simulink model "full_simulation_split_hil_new_connection"  (Simulink 7.9)
settings: Solver=ode1  StartTime=0  StopTime=10  FixedStep=Ts  RelTol=1e-8
values from neighbouring files (symbols this model uses):
  A_fx = 2e-2 * 0.4    (= 0.008)    [QR_DI_Init.m]    (also in quadro_cascade_disturbance_wo_wind.m)
  A_fy = A_fx    (= 0.008)    [QR_DI_Init.m]    (also in quadro_cascade_disturbance_wo_wind.m)
  A_fz = 2 * A_fx    (= 0.016)    [QR_DI_Init.m]    (also in quadro_cascade_disturbance_wo_wind.m)
  Bias_Phi = -0.0088    [QR_DI_Init.m]    (also in Reference_Calibration.m = mean(Phi))
  Bias_Theta = 0.022    [QR_DI_Init.m]    (also in Reference_Calibration.m = mean(Theta))
  command_on = 1    [QR_DI_Init.m]    (also in quadro_cascade_disturbance_wo_wind.m)
  cw_x = 1.05    [QR_DI_Init.m]    (also in quadro_cascade_disturbance_wo_wind.m)
  cw_y = cw_x    (= 1.05)    [QR_DI_Init.m]    (also in quadro_cascade_disturbance_wo_wind.m)
  cw_z = 1.05    [QR_DI_Init.m]    (also in quadro_cascade_disturbance_wo_wind.m)
  deltaTm = 0.2    [QR_DI_Init.m]    (also in quadro_cascade_disturbance_wo_wind.m)
  den_psi_ref = poly( ones(1,2) * -1 * T_psi_ref)    [QR_DI_Init.m]    (also in quadro_cascade_disturbance_wo_wind.m)
  den_x_ref = poly( ones(1,4) * -1 * T_x_ref)    [QR_DI_Init.m]    (also in quadro_cascade_disturbance_wo_wind.m)
  den_y_ref = poly( ones(1,4) * -1 * T_y_ref)    [QR_DI_Init.m]    (also in quadro_cascade_disturbance_wo_wind.m)
  den_z_ref = poly( ones(1,4) * -1 * T_z_ref)    [QR_DI_Init.m]    (also in quadro_cascade_disturbance_wo_wind.m)
  drot = 0.0117    [QR_DI_Init.m]    (also in quadro_cascade_disturbance_wo_wind.m = 0.2)
  dtran = 0.01    [QR_DI_Init.m]    (also in quadro_cascade_disturbance_wo_wind.m = 0.003)
  Fz_gain = 1 + 0.05*rand(1)    [QR_DI_Init.m]    (also in quadro_cascade_disturbance_wo_wind.m)
  Fz_lo = - 1.2 * m * g    (= -3.5316)    [QR_DI_Init.m]    (also in quadro_cascade_disturbance_wo_wind.m = -4.1202)
  Fz_up = 0    [QR_DI_Init.m]    (also in quadro_cascade_disturbance_wo_wind.m)
  g = 9.81    [QR_DI_Init.m]    (also in quadro_cascade_disturbance_wo_wind.m)
  Iq = [I_xx 0 0 ; 0 I_yy 0 ; 0 0 I_zz ]    [QR_DI_Init.m]    (also in quadro_cascade_disturbance_wo_wind.m = [0.0605 0 0; 0 0.0605 0; 0 0 0.018])
  K_err = old(:,2:end)    [QR_DI_Init.m]    (also in quadro_cascade_disturbance_wo_wind.m)
  K_Mot_Force = 0.3512    [QR_DI_Init.m]    (also in quadro_cascade_disturbance_wo_wind.m)
  K_Mot_Torque = 0.013    [QR_DI_Init.m]    (also in quadro_cascade_disturbance_wo_wind.m = 0.0013)
  l = 0.25    [QR_DI_Init.m]    (also in quadro_cascade_disturbance_wo_wind.m = 0.2775)
  m = 0.30    (= 0.3)    [QR_DI_Init.m]    (also in quadro_cascade_disturbance_wo_wind.m)
  m_real = m * ( 1 + 0.05*rand(1))    [QR_DI_Init.m]    (also in quadro_cascade_disturbance_wo_wind.m)
  Mm = 0.0    (= 0)    [QR_DI_Init.m]    (also in quadro_cascade_disturbance_wo_wind.m = 0.5)
  Mx_lo = - Mx_up    (= -0.2)    [QR_DI_Init.m]    (also in quadro_cascade_disturbance_wo_wind.m)
  Mx_up = 0.20    (= 0.2)    [QR_DI_Init.m]    (also in quadro_cascade_disturbance_wo_wind.m)
  My_lo = - My_up    (= -0.2)    [QR_DI_Init.m]    (also in quadro_cascade_disturbance_wo_wind.m)
  My_up = 0.20    (= 0.2)    [QR_DI_Init.m]    (also in quadro_cascade_disturbance_wo_wind.m)
  Mz_lo = - Mz_up    (= -0.02)    [QR_DI_Init.m]    (also in quadro_cascade_disturbance_wo_wind.m = -0.002)
  Mz_up = 0.02    [QR_DI_Init.m]    (also in quadro_cascade_disturbance_wo_wind.m = 0.002)
  phase_wind_z = 0    [QR_DI_Init.m]    (also in quadro_cascade_disturbance_wo_wind.m)
  psi_p_lim = 10*pi/180    (= 0.174532925199)    [QR_DI_Init.m]    (also in quadro_cascade_disturbance_wo_wind.m = 5)
  PWM_MAX = 200    [QR_DI_Init.m]    (also in quadro_cascade_disturbance_wo_wind.m)
  rho_air = 1.2041    [QR_DI_Init.m]    (also in quadro_cascade_disturbance_wo_wind.m)
  sample_time_noise_psi = 0.1    [QR_DI_Init.m]
  sample_time_noise_x = 0.2    [QR_DI_Init.m]
  sample_time_noise_y = 0.2    [QR_DI_Init.m]
  sample_time_noise_z = 0.1    [QR_DI_Init.m]
  seed_psi = seedvector(7)    [QR_DI_Init.m]
  seed_x = seedvector(1)    [QR_DI_Init.m]    (also in quadro_cascade_disturbance_wo_wind.m)
  seed_xp = seedvector(4)    [QR_DI_Init.m]    (also in quadro_cascade_disturbance_wo_wind.m)
  seed_y = seedvector(2)    [QR_DI_Init.m]    (also in quadro_cascade_disturbance_wo_wind.m)
  seed_yp = seedvector(5)    [QR_DI_Init.m]    (also in quadro_cascade_disturbance_wo_wind.m)
  seed_z = seedvector(3)    [QR_DI_Init.m]    (also in quadro_cascade_disturbance_wo_wind.m)
  seed_zp = seedvector(6)    [QR_DI_Init.m]    (also in quadro_cascade_disturbance_wo_wind.m)
  std_dev_psi = 1 * pi/180 * Noise_on    (= 0)    [QR_DI_Init.m]
  std_dev_x = 1e-1 * Noise_on    (= 0)    [QR_DI_Init.m]
  std_dev_xp = 0.03 * Noise_on    (= 0)    [QR_DI_Init.m]
  std_dev_y = 1e-1 * Noise_on    (= 0)    [QR_DI_Init.m]
  std_dev_yp = 0.03 * Noise_on    (= 0)    [QR_DI_Init.m]
  std_dev_z = 0.03 * Noise_on    (= 0)    [QR_DI_Init.m]
  std_dev_zp = 0.03 * Noise_on    (= 0)    [QR_DI_Init.m]
  T_refalt = 0.01    [QR_DI_Init.m]    (also in quadro_cascade_disturbance_wo_wind.m)
  T_wind_z = 24    [QR_DI_Init.m]    (also in quadro_cascade_disturbance_wo_wind.m)
  Tm = 10    [QR_DI_Init.m]    (also in quadro_cascade_disturbance_wo_wind.m)
  Ts = 1e-2    (= 0.01)    [QR_DI_Init.m]    (also in quadro_cascade_disturbance_wo_wind.m)
  v_wind_max_z = 2    [QR_DI_Init.m]    (also in quadro_cascade_disturbance_wo_wind.m)
  wind_on = 0    [QR_DI_Init.m]    (also in quadro_cascade_disturbance_wo_wind.m)
  x_p_lim = 1.5    [QR_DI_Init.m]    (also in quadro_cascade_disturbance_wo_wind.m = 5)
  y_p_lim = 1.5    [QR_DI_Init.m]    (also in quadro_cascade_disturbance_wo_wind.m = 5)
  z_p_lim = 1    [QR_DI_Init.m]    (also in quadro_cascade_disturbance_wo_wind.m = 1.5)
undefined symbols (not defined in the file or in its folder): T_wind_fine, v_wind_x_fine, v_wind_y_fine
libraries: simulink x5, dspsigops x4, Ports x4, aerolibtransform2 x3, dspmtrx3 x1, aerolibutil x1
(part 4 of 6)

== matlab function Dynamic Inversion of the Extended System/bx1/Embedded MATLAB Function1 ==
  data: xwhole_ext input double size=[14 1]; bx output double size=[4 1]; m_in input double; I input double size=[3 3]; dtran input double; drot input double

% S.H. 26.03.2013
% correct bx

function bx = fcn(xwhole_ext, m_in, I, dtran, drot)
% This block supports the Embedded MATLAB subset.
% See the help menu for details. 
x = xwhole_ext(1);
y = xwhole_ext(2);
z = xwhole_ext(3);
dx = xwhole_ext(4);
dy = xwhole_ext(5);
dz = xwhole_ext(6);

phi = xwhole_ext(7);
theta = xwhole_ext(8);
psi = xwhole_ext(9);
p = xwhole_ext(10);
q = xwhole_ext(11);
r = xwhole_ext(12);


xi1 = xwhole_ext(13) +eps;
dxi1 = xwhole_ext(14) +eps;


%g = -9.81;
g = -9.81;   % S.H. 26.03.2013

m = m_in;

% FIXME: the bx is still the one without deviation components
Ixx = I(1,1);
Ixy = I(1,2);
Ixz = I(1,3);
Iyy = I(2,2);
Iyz = I(2,3);
Izz = I(3,3);

% S.H. 26.03.2013
bx =    [...
(p + r*cos(phi)*tan(theta) + q*sin(phi)*tan(theta))*((dxi1*(cos(phi)*sin(psi) - cos(psi)*sin(phi)*sin(theta)))/m - (xi1*(sin(phi)*sin(psi) + cos(phi)*cos(psi)*sin(theta))*(p + r*cos(phi)*tan(theta) + q*sin(phi)*tan(theta)))/m + (xi1*((r*cos(phi))/cos(theta) + (q*sin(phi))/cos(theta))*(cos(phi)*cos(psi) + sin(phi)*sin(psi)*sin(theta)))/m + (xi1*((q*cos(phi))/cos(theta) - (r*sin(phi))/cos(theta))*(cos(psi)*sin(phi) - cos(phi)*sin(psi)*sin(theta)))/m - (dtran*xi1*(cos(phi)*sin(psi) - cos(psi)*sin(phi)*sin(theta)))/m^2 + (xi1*(cos(phi)*sin(psi) - cos(psi)*sin(phi)*sin(theta))*(q*cos(phi)*tan(theta) - r*sin(phi)*tan(theta)))/m - (xi1*cos(phi)*cos(psi)*cos(theta)*(r*cos(phi) + q*sin(phi)))/m - (xi1*cos(psi)*cos(theta)*sin(phi)*(q*cos(phi) - r*sin(phi)))/m) - ((Ixx*p*r - Izz*p*r)/Iyy + (drot*q)/Iyy)*((xi1*sin(phi)*(cos(psi)*sin(phi) - cos(phi)*sin(psi)*sin(theta)))/(m*cos(theta)) + (xi1*cos(phi)^2*cos(psi)*cos(theta))/m + (xi1*sin(phi)*tan(theta)*(cos(phi)*sin(psi) - cos(psi)*sin(phi)*sin(theta)))/m) + ((Ixx*p*q - Iyy*p*q)/Izz - (drot*r)/Izz)*((xi1*cos(phi)*(cos(psi)*sin(phi) - cos(phi)*sin(psi)*sin(theta)))/(m*cos(theta)) + (xi1*cos(phi)*tan(theta)*(cos(phi)*sin(psi) - cos(psi)*sin(phi)*sin(theta)))/m - (xi1*cos(phi)*cos(psi)*cos(theta)*sin(phi))/m) - ((r*cos(phi))/cos(theta) + (q*sin(phi))/cos(theta))*((xi1*((r*cos(phi))/cos(theta) + (q*sin(phi))/cos(theta))*(sin(phi)*sin(psi) + cos(phi)*cos(psi)*sin(theta)))/m - (xi1*(cos(phi)*cos(psi) + sin(phi)*sin(psi)*sin(theta))*(p + r*cos(phi)*tan(theta) + q*sin(phi)*tan(theta)))/m - (dxi1*(cos(psi)*sin(phi) - cos(phi)*sin(psi)*sin(theta)))/m + (dtran*xi1*(cos(psi)*sin(phi) - cos(phi)*sin(psi)*sin(theta)))/m^2 + (xi1*cos(phi)*cos(theta)*sin(psi)*(q*cos(phi) - r*sin(phi)))/m) - (q*cos(phi) - r*sin(phi))*((xi1*cos(psi)*cos(theta)*sin(phi)*(p + r*cos(phi)*tan(theta) + q*sin(phi)*tan(theta)))/m - (xi1*(r*cos(phi)*(tan(theta)^2 + 1) + q*sin(phi)*(tan(theta)^2 + 1))*(cos(phi)*sin(psi) - cos(psi)*sin(phi)*sin(theta)))/m - (dxi1*cos(phi)*cos(psi)*cos(theta))/m - (xi1*(cos(psi)*sin(phi) - cos(phi)*sin(psi)*sin(theta))*((r*cos(phi)*sin(theta))/cos(theta)^2 + (q*sin(phi)*sin(theta))/cos(theta)^2))/m + (xi1*cos(phi)*cos(theta)*sin(psi)*((r*cos(phi))/cos(theta) + (q*sin(phi))/cos(theta)))/m + (dtran*xi1*cos(phi)*cos(psi)*cos(theta))/m^2 + (xi1*cos(phi)*cos(psi)*sin(theta)*(q*cos(phi) - r*sin(phi)))/m) + dxi1*(((cos(phi)*sin(psi) - cos(psi)*sin(phi)*sin(theta))*(p + r*cos(phi)*tan(theta) + q*sin(phi)*tan(theta)))/m - (dtran*(sin(phi)*sin(psi) + cos(phi)*cos(psi)*sin(theta)))/m^2 + (((r*cos(phi))/cos(theta) + (q*sin(phi))/cos(theta))*(cos(psi)*sin(phi) - cos(phi)*sin(psi)*sin(theta)))/m + (cos(phi)*cos(psi)*cos(theta)*(q*cos(phi) - r*sin(phi)))/m) + (dtran^2*((xi1*(sin(phi)*sin(psi) + cos(phi)*cos(psi)*sin(theta)))/m - (dtran*dx)/m))/m^2 + (xi1*(cos(phi)*sin(psi) - cos(psi)*sin(phi)*sin(theta))*((Iyy*q*r - Izz*q*r)/Ixx - (drot*p)/Ixx))/m;
        dxi1*((dtran*(cos(psi)*sin(phi) - cos(phi)*sin(psi)*sin(theta)))/m^2 - ((cos(phi)*cos(psi) + sin(phi)*sin(psi)*sin(theta))*(p + r*cos(phi)*tan(theta) + q*sin(phi)*tan(theta)))/m + (((r*cos(phi))/cos(theta) + (q*sin(phi))/cos(theta))*(sin(phi)*sin(psi) + cos(phi)*cos(psi)*sin(theta)))/m + (cos(phi)*cos(theta)*sin(psi)*(q*cos(phi) - r*sin(phi)))/m) - ((Ixx*p*r - Izz*p*r)/Iyy + (drot*q)/Iyy)*((xi1*sin(phi)*(sin(phi)*sin(psi) + cos(phi)*cos(psi)*sin(theta)))/(m*cos(theta)) + (xi1*cos(phi)^2*cos(theta)*sin(psi))/m - (xi1*sin(phi)*tan(theta)*(cos(phi)*cos(psi) + sin(phi)*sin(psi)*sin(theta)))/m) - (p + r*cos(phi)*tan(theta) + q*sin(phi)*tan(theta))*((dxi1*(cos(phi)*cos(psi) + sin(phi)*sin(psi)*sin(theta)))/m - (xi1*(cos(psi)*sin(phi) - cos(phi)*sin(psi)*sin(theta))*(p + r*cos(phi)*tan(theta) + q*sin(phi)*tan(theta)))/m - (xi1*((r*cos(phi))/cos(theta) + (q*sin(phi))/cos(theta))*(cos(phi)*sin(psi) - cos(psi)*sin(phi)*sin(theta)))/m - (xi1*((q*cos(phi))/cos(theta) - (r*sin(phi))/cos(theta))*(sin(phi)*sin(psi) + cos(phi)*cos(psi)*sin(theta)))/m - (dtran*xi1*(cos(phi)*cos(psi) + sin(phi)*sin(psi)*sin(theta)))/m^2 + (xi1*(cos(phi)*cos(psi) + sin(phi)*sin(psi)*sin(theta))*(q*cos(phi)*tan(theta) - r*sin(phi)*tan(theta)))/m + (xi1*cos(phi)*cos(theta)*sin(psi)*(r*cos(phi) + q*sin(phi)))/m + (xi1*cos(theta)*sin(phi)*sin(psi)*(q*cos(phi) - r*sin(phi)))/m) - ((Ixx*p*q - Iyy*p*q)/Izz - (drot*r)/Izz)*((xi1*cos(phi)*tan(theta)*(cos(phi)*cos(psi) + sin(phi)*sin(psi)*sin(theta)))/m - (xi1*cos(phi)*(sin(phi)*sin(psi) + cos(phi)*cos(psi)*sin(theta)))/(m*cos(theta)) + (xi1*cos(phi)*cos(theta)*sin(phi)*sin(psi))/m) + ((r*cos(phi))/cos(theta) + (q*sin(phi))/cos(theta))*((dxi1*(sin(phi)*sin(psi) + cos(phi)*cos(psi)*sin(theta)))/m + (xi1*(cos(phi)*sin(psi) - cos(psi)*sin(phi)*sin(theta))*(p + r*cos(phi)*tan(theta) + q*sin(phi)*tan(theta)))/m + (xi1*((r*cos(phi))/cos(theta) + (q*sin(phi))/cos(theta))*(cos(psi)*sin(phi) - cos(phi)*sin(psi)*sin(theta)))/m - (dtran*xi1*(sin(phi)*sin(psi) + cos(phi)*cos(psi)*sin(theta)))/m^2 + (xi1*cos(phi)*cos(psi)*cos(theta)*(q*cos(phi) - r*sin(phi)))/m) - (q*cos(phi) - r*sin(phi))*((xi1*(r*cos(phi)*(tan(theta)^2 + 1) + q*sin(phi)*(tan(theta)^2 + 1))*(cos(phi)*cos(psi) + sin(phi)*sin(psi)*sin(theta)))/m - (xi1*(sin(phi)*sin(psi) + cos(phi)*cos(psi)*sin(theta))*((r*cos(phi)*sin(theta))/cos(theta)^2 + (q*sin(phi)*sin(theta))/cos(theta)^2))/m - (dxi1*cos(phi)*cos(theta)*sin(psi))/m + (xi1*cos(theta)*sin(phi)*sin(psi)*(p + r*cos(phi)*tan(theta) + q*sin(phi)*tan(theta)))/m - (xi1*cos(phi)*cos(psi)*cos(theta)*((r*cos(phi))/cos(theta) + (q*sin(phi))/cos(theta)))/m + (dtran*xi1*cos(phi)*cos(theta)*sin(psi))/m^2 + (xi1*cos(phi)*sin(psi)*sin(theta)*(q*cos(phi) - r*sin(phi)))/m) - (dtran^2*((xi1*(cos(psi)*sin(phi) - cos(phi)*sin(psi)*sin(theta)))/m + (dtran*dy)/m))/m^2 - (xi1*(cos(phi)*cos(psi) + sin(phi)*sin(psi)*sin(theta))*((Iyy*q*r - Izz*q*r)/Ixx - (drot*p)/Ixx))/m;
        ((Ixx*p*q - Iyy*p*q)/Izz - (drot*r)/Izz)*((xi1*cos(phi)*sin(phi)*sin(theta))/m - (xi1*cos(phi)*cos(theta)*sin(phi)*tan(theta))/m) - (q*cos(phi) - r*sin(phi))*((dxi1*cos(phi)*sin(theta))/m + (xi1*cos(phi)*cos(theta)*(q*cos(phi) - r*sin(phi)))/m + (xi1*cos(theta)*sin(phi)*(r*cos(phi)*(tan(theta)^2 + 1) + q*sin(phi)*(tan(theta)^2 + 1)))/m - (xi1*sin(phi)*sin(theta)*(p + r*cos(phi)*tan(theta) + q*sin(phi)*tan(theta)))/m - (dtran*xi1*cos(phi)*sin(theta))/m^2) - (p + r*cos(phi)*tan(theta) + q*sin(phi)*tan(theta))*((dxi1*cos(theta)*sin(phi))/m - (xi1*cos(phi)*sin(theta)*(r*cos(phi) + q*sin(phi)))/m - (xi1*sin(phi)*sin(theta)*(q*cos(phi) - r*sin(phi)))/m + (xi1*cos(phi)*cos(theta)*(p + r*cos(phi)*tan(theta) + q*sin(phi)*tan(theta)))/m - (dtran*xi1*cos(theta)*sin(phi))/m^2 + (xi1*cos(theta)*sin(phi)*(q*cos(phi)*tan(theta) - r*sin(phi)*tan(theta)))/m) + ((Ixx*p*r - Izz*p*r)/Iyy + (drot*q)/Iyy)*((xi1*cos(phi)^2*sin(theta))/m + (xi1*cos(theta)*sin(phi)^2*tan(theta))/m) - dxi1*((dtran*cos(phi)*cos(theta))/m^2 + (cos(phi)*sin(theta)*(q*cos(phi) - r*sin(phi)))/m + (cos(theta)*sin(phi)*(p + r*cos(phi)*tan(theta) + q*sin(phi)*tan(theta)))/m) + (dtran^2*(g - (dtran*dz)/m + (xi1*cos(phi)*cos(theta))/m))/m^2 - (xi1*cos(theta)*sin(phi)*((Iyy*q*r - Izz*q*r)/Ixx - (drot*p)/Ixx))/m;
        (q*cos(phi) - r*sin(phi))*((r*cos(phi)*sin(theta))/cos(theta)^2 + (q*sin(phi)*sin(theta))/cos(theta)^2) + ((q*cos(phi))/cos(theta) - (r*sin(phi))/cos(theta))*(p + r*cos(phi)*tan(theta) + q*sin(phi)*tan(theta)) + (cos(phi)*((Ixx*p*q - Iyy*p*q)/Izz - (drot*r)/Izz))/cos(theta) - (sin(phi)*((Ixx*p*r - Izz*p*r)/Iyy + (drot*q)/Iyy))/cos(theta)];
 
               
    
%% Old    
    
% 
% function bx = fcn(xwhole_ext, m_in, I, dtran, drot)
% % This block supports the Embedded MATLAB subset.
% % See the help menu for details. 
% x = xwhole_ext(1);
% y = xwhole_ext(2);
% z = xwhole_ext(3);
% dx = xwhole_ext(4);
% dy = xwhole_ext(5);
% dz = xwhole_ext(6);
% 
% phi = xwhole_ext(7);
% theta = xwhole_ext(8);
% psi = xwhole_ext(9);
% p = xwhole_ext(10);
% q = xwhole_ext(11);
% r = xwhole_ext(12);
% 
% 
% xi1 = xwhole_ext(13) +eps;
% dxi1 = xwhole_ext(14) +eps;
% 
% 
% g = -9.81;
% 
% m = m_in;
% 
% % FIXME: the bx is still the one without deviation components
% Ixx = I(1,1);
% Ixy = I(1,2);
% Ixz = I(1,3);
% Iyy = I(2,2);
% Iyz = I(2,3);
% Izz = I(3,3);
% 
% % bx = [...
% % -dtran^3*(-dtran*dx+xi1/m*(sin(psi)*sin(phi)+cos(psi)*cos(phi)*sin(theta)))+(dtran^2*xi1/m*(sin(psi)*cos(phi)-cos(psi)*sin(phi)*sin(theta))+(-dtran*xi1/m*(-sin(psi)*sin(phi)-cos(psi)*cos(phi)*sin(theta))+xi1/m*(cos(psi)*sin(phi)*sin(theta)-sin(psi)*cos(phi))*(p+sin(phi)*tan(theta)*q+cos(phi)*tan(theta)*r)+2*xi1/m*(-sin(psi)*sin(phi)-cos(psi)*cos(phi)*sin(theta))*(cos(phi)*tan(theta)*q-sin(phi)*tan(theta)*r)+xi1/m*(sin(psi)*cos(phi)-cos(psi)*sin(phi)*sin(theta))*(-sin(phi)*tan(theta)*q-cos(phi)*tan(theta)*r)-xi1/m*cos(psi)*cos(phi)*cos(theta)*(cos(phi)*q-sin(phi)*r)-2*xi1/m*cos(psi)*sin(phi)*cos(theta)*(-sin(phi)*q-cos(phi)*r)+xi1/m*cos(psi)*cos(phi)*cos(theta)*(-cos(phi)*q+sin(phi)*r)+xi1/m*(cos(phi)*sin(psi)*sin(theta)-cos(psi)*sin(phi))*(sin(phi)/cos(theta)*q+cos(phi)/cos(theta)*r)+2*xi1/m*(cos(psi)*cos(phi)+sin(phi)*sin(psi)*sin(theta))*(cos(phi)/cos(theta)*q-sin(phi)/cos(theta)*r)+xi1/m*(-cos(phi)*sin(psi)*sin(theta)+cos(psi)*sin(phi))*(-sin(phi)/cos(theta)*q-cos(phi)/cos(theta)*r)+1/m*(-sin(psi)*sin(phi)-cos(psi)*cos(phi)*sin(theta))*dxi1)*(p+sin(phi)*tan(theta)*q+cos(phi)*tan(theta)*r)+(-dtran*xi1/m*(sin(psi)*cos(phi)-cos(psi)*sin(phi)*sin(theta))+xi1/m*(-sin(psi)*sin(phi)-cos(psi)*cos(phi)*sin(theta))*(p+sin(phi)*tan(theta)*q+cos(phi)*tan(theta)*r)+xi1/m*(sin(psi)*cos(phi)-cos(psi)*sin(phi)*sin(theta))*(cos(phi)*tan(theta)*q-sin(phi)*tan(theta)*r)-xi1/m*cos(psi)*sin(phi)*cos(theta)*(cos(phi)*q-sin(phi)*r)+xi1/m*cos(psi)*cos(phi)*cos(theta)*(-sin(phi)*q-cos(phi)*r)+xi1/m*(cos(psi)*cos(phi)+sin(phi)*sin(psi)*sin(theta))*(sin(phi)/cos(theta)*q+cos(phi)/cos(theta)*r)+xi1/m*(-cos(phi)*sin(psi)*sin(theta)+cos(psi)*sin(phi))*(cos(phi)/cos(theta)*q-sin(phi)/cos(theta)*r)+1/m*(sin(psi)*cos(phi)-cos(psi)*sin(phi)*sin(theta))*dxi1)*(cos(phi)*tan(theta)*q-sin(phi)*tan(theta)*r)+(dtran*xi1/m*cos(psi)*sin(phi)*cos(theta)-xi1/m*cos(psi)*cos(phi)*cos(theta)*(p+sin(phi)*tan(theta)*q+cos(phi)*tan(theta)*r)-xi1/m*cos(psi)*sin(phi)*cos(theta)*(cos(phi)*tan(theta)*q-sin(phi)*tan(theta)*r)+xi1/m*(-sin(psi)*sin(phi)-cos(psi)*cos(phi)*sin(theta))*(sin(phi)*(1+tan(theta)^2)*q+cos(phi)*(1+tan(theta)^2)*r)+xi1/m*(sin(psi)*cos(phi)-cos(psi)*sin(phi)*sin(theta))*(cos(phi)*(1+tan(theta)^2)*q-sin(phi)*(1+tan(theta)^2)*r)+xi1/m*cos(psi)*sin(phi)*sin(theta)*(cos(phi)*q-sin(phi)*r)-xi1/m*cos(psi)*cos(phi)*sin(theta)*(-sin(phi)*q-cos(phi)*r)+xi1/m*sin(phi)*sin(psi)*cos(theta)*(sin(phi)/cos(theta)*q+cos(phi)/cos(theta)*r)-xi1/m*cos(phi)*sin(psi)*cos(theta)*(cos(phi)/cos(theta)*q-sin(phi)/cos(theta)*r)+xi1/m*(cos(psi)*cos(phi)+sin(phi)*sin(psi)*sin(theta))*(sin(phi)/cos(theta)^2*q*sin(theta)+cos(phi)/cos(theta)^2*r*sin(theta))+xi1/m*(-cos(phi)*sin(psi)*sin(theta)+cos(psi)*sin(phi))*(cos(phi)/cos(theta)^2*q*sin(theta)-sin(phi)/cos(theta)^2*r*sin(theta))-1/m*cos(psi)*sin(phi)*cos(theta)*dxi1)*(cos(phi)*q-sin(phi)*r)+(-dtran*xi1/m*cos(psi)*cos(phi)*cos(theta)-xi1/m*cos(psi)*sin(phi)*cos(theta)*(p+sin(phi)*tan(theta)*q+cos(phi)*tan(theta)*r)+xi1/m*(sin(psi)*cos(phi)-cos(psi)*sin(phi)*sin(theta))*(sin(phi)*(1+tan(theta)^2)*q+cos(phi)*(1+tan(theta)^2)*r)-xi1/m*cos(psi)*cos(phi)*sin(theta)*(cos(phi)*q-sin(phi)*r)-xi1/m*cos(phi)*sin(psi)*cos(theta)*(sin(phi)/cos(theta)*q+cos(phi)/cos(theta)*r)+xi1/m*(-cos(phi)*sin(psi)*sin(theta)+cos(psi)*sin(phi))*(sin(phi)/cos(theta)^2*q*sin(theta)+cos(phi)/cos(theta)^2*r*sin(theta))+1/m*cos(psi)*cos(phi)*cos(theta)*dxi1)*(-sin(phi)*q-cos(phi)*r)+(-dtran*xi1/m*(cos(psi)*cos(phi)+sin(phi)*sin(psi)*sin(theta))+xi1/m*(cos(phi)*sin(psi)*sin(theta)-cos(psi)*sin(phi))*(p+sin(phi)*tan(theta)*q+cos(phi)*tan(theta)*r)+xi1/m*(cos(psi)*cos(phi)+sin(phi)*sin(psi)*sin(theta))*(cos(phi)*tan(theta)*q-sin(phi)*tan(theta)*r)+xi1/m*sin(psi)*sin(phi)*cos(theta)*(cos(phi)*q-sin(phi)*r)-xi1/m*sin(psi)*cos(phi)*cos(theta)*(-sin(phi)*q-cos(phi)*r)+xi1/m*(cos(psi)*sin(phi)*sin(theta)-sin(psi)*cos(phi))*(sin(phi)/cos(theta)*q+cos(phi)/cos(theta)*r)+xi1/m*(-sin(psi)*sin(phi)-cos(psi)*cos(phi)*sin(theta))*(cos(phi)/cos(theta)*q-sin(phi)/cos(theta)*r)+1/m*(cos(psi)*cos(phi)+sin(phi)*sin(psi)*sin(theta))*dxi1)*(sin(phi)/cos(theta)*q+cos(phi)/cos(theta)*r)+(-dtran*xi1/m*(-cos(phi)*sin(psi)*sin(theta)+cos(psi)*sin(phi))+xi1/m*(cos(psi)*cos(phi)+sin(phi)*sin(psi)*sin(theta))*(p+sin(phi)*tan(theta)*q+cos(phi)*tan(theta)*r)-xi1/m*sin(psi)*cos(phi)*cos(theta)*(cos(phi)*q-sin(phi)*r)+xi1/m*(-sin(psi)*sin(phi)-cos(psi)*cos(phi)*sin(theta))*(sin(phi)/cos(theta)*q+cos(phi)/cos(theta)*r)+1/m*(-cos(phi)*sin(psi)*sin(theta)+cos(psi)*sin(phi))*dxi1)*(cos(phi)/cos(theta)*q-sin(phi)/cos(theta)*r)+xi1/m*(-sin(psi)*sin(phi)-cos(psi)*cos(phi)*sin(theta))*(-drot*p-1/Ixx*(q*Izz*r-r*Iyy*q)+xi2/Ixx)+(xi1/m*(-sin(psi)*sin(phi)-cos(psi)*cos(phi)*sin(theta))*sin(phi)*tan(theta)+xi1/m*(sin(psi)*cos(phi)-cos(psi)*sin(phi)*sin(theta))*cos(phi)*tan(theta)-2*xi1/m*cos(phi)*cos(psi)*cos(theta)*sin(phi)+xi1/m*(cos(psi)*cos(phi)+sin(phi)*sin(psi)*sin(theta))*sin(phi)/cos(theta)+xi1/m*(-cos(phi)*sin(psi)*sin(theta)+cos(psi)*sin(phi))*cos(phi)/cos(theta))*(-drot*q-1/Iyy*(r*Ixx*p-p*Izz*r)+xi3/Iyy)+(xi1/m*(-sin(psi)*sin(phi)-cos(psi)*cos(phi)*sin(theta))*cos(phi)*tan(theta)-xi1/m*(sin(psi)*cos(phi)-cos(psi)*sin(phi)*sin(theta))*sin(phi)*tan(theta)+xi1/m*sin(phi)^2*cos(psi)*cos(theta)-xi1/m*cos(phi)^2*cos(psi)*cos(theta)+xi1/m*(cos(psi)*cos(phi)+sin(phi)*sin(psi)*sin(theta))*cos(phi)/cos(theta)-xi1/m*(-cos(phi)*sin(psi)*sin(theta)+cos(psi)*sin(phi))*sin(phi)/cos(theta))*(-drot*r-1/Izz*(p*Iyy*q-q*Ixx*p)+xi4/Izz)+(-dtran/m*(sin(psi)*cos(phi)-cos(psi)*sin(phi)*sin(theta))+1/m*(-sin(psi)*sin(phi)-cos(psi)*cos(phi)*sin(theta))*(p+sin(phi)*tan(theta)*q+cos(phi)*tan(theta)*r)+1/m*(sin(psi)*cos(phi)-cos(psi)*sin(phi)*sin(theta))*(cos(phi)*tan(theta)*q-sin(phi)*tan(theta)*r)-1/m*cos(psi)*sin(phi)*cos(theta)*(cos(phi)*q-sin(phi)*r)+1/m*cos(psi)*cos(phi)*cos(theta)*(-sin(phi)*q-cos(phi)*r)+1/m*(cos(psi)*cos(phi)+sin(phi)*sin(psi)*sin(theta))*(sin(phi)/cos(theta)*q+cos(phi)/cos(theta)*r)+1/m*(-cos(phi)*sin(psi)*sin(theta)+cos(psi)*sin(phi))*(cos(phi)/cos(theta)*q-sin(phi)/cos(theta)*r))*dxi1+1/m*(sin(psi)*cos(phi)-cos(psi)*sin(phi)*sin(theta))*ddxi1)*(p+sin(phi)*tan(theta)*q+cos(phi)*tan(theta)*r)+(dtran^2*xi1/m*cos(psi)*cos(phi)*cos(theta)+(dtran*xi1/m*cos(psi)*sin(phi)*cos(theta)-xi1/m*cos(psi)*cos(phi)*cos(theta)*(p+sin(phi)*tan(theta)*q+cos(phi)*tan(theta)*r)-xi1/m*cos(psi)*sin(phi)*cos(theta)*(cos(phi)*tan(theta)*q-sin(phi)*tan(theta)*r)+xi1/m*(-sin(psi)*sin(phi)-cos(psi)*cos(phi)*sin(theta))*(sin(phi)*(1+tan(theta)^2)*q+cos(phi)*(1+tan(theta)^2)*r)+xi1/m*(sin(psi)*cos(phi)-cos(psi)*sin(phi)*sin(theta))*(cos(phi)*(1+tan(theta)^2)*q-sin(phi)*(1+tan(theta)^2)*r)+xi1/m*cos(psi)*sin(phi)*sin(theta)*(cos(phi)*q-sin(phi)*r)-xi1/m*cos(psi)*cos(phi)*sin(theta)*(-sin(phi)*q-cos(phi)*r)+xi1/m*sin(phi)*sin(psi)*cos(theta)*(sin(phi)/cos(theta)*q+cos(phi)/cos(theta)*r)-xi1/m*cos(phi)*sin(psi)*cos(theta)*(cos(phi)/cos(theta)*q-sin(phi)/cos(theta)*r)+xi1/m*(cos(psi)*cos(phi)+sin(phi)*sin(psi)*sin(theta))*(sin(phi)/cos(theta)^2*q*sin(theta)+cos(phi)/cos(theta)^2*r*sin(theta))+xi1/m*(-cos(phi)*sin(psi)*sin(theta)+cos(psi)*sin(phi))*(cos(phi)/cos(theta)^2*q*sin(theta)-sin(phi)/cos(theta)^2*r*sin(theta))-1/m*cos(psi)*sin(phi)*cos(theta)*dxi1)*(p+sin(phi)*tan(theta)*q+cos(phi)*tan(theta)*r)+(-dtran*xi1/m*(sin(psi)*cos(phi)-cos(psi)*sin(phi)*sin(theta))+xi1/m*(-sin(psi)*sin(phi)-cos(psi)*cos(phi)*sin(theta))*(p+sin(phi)*tan(theta)*q+cos(phi)*tan(theta)*r)+xi1/m*(sin(psi)*cos(phi)-cos(psi)*sin(phi)*sin(theta))*(cos(phi)*tan(theta)*q-sin(phi)*tan(theta)*r)-xi1/m*cos(psi)*sin(phi)*cos(theta)*(cos(phi)*q-sin(phi)*r)+xi1/m*cos(psi)*cos(phi)*cos(theta)*(-sin(phi)*q-cos(phi)*r)+xi1/m*(cos(psi)*cos(phi)+sin(phi)*sin(psi)*sin(theta))*(sin(phi)/cos(theta)*q+cos(phi)/cos(theta)*r)+xi1/m*(-cos(phi)*sin(psi)*sin(theta)+cos(psi)*sin(phi))*(cos(phi)/cos(theta)*q-sin(phi)/cos(theta)*r)+1/m*(sin(psi)*cos(phi)-cos(psi)*sin(phi)*sin(theta))*dxi1)*(sin(phi)*(1+tan(theta)^2)*q+cos(phi)*(1+tan(theta)^2)*r)+(dtran*xi1/m*cos(psi)*cos(phi)*sin(theta)+xi1/m*cos(psi)*sin(phi)*sin(theta)*(p+sin(phi)*tan(theta)*q+cos(phi)*tan(theta)*r)-2*xi1/m*cos(psi)*sin(phi)*cos(theta)*(sin(phi)*(1+tan(theta)^2)*q+cos(phi)*(1+tan(theta)^2)*r)+xi1/m*(sin(psi)*cos(phi)-cos(psi)*sin(phi)*sin(theta))*(2*sin(phi)*tan(theta)*(1+tan(theta)^2)*q+2*cos(phi)*tan(theta)*(1+tan(theta)^2)*r)-xi1/m*cos(psi)*cos(phi)*cos(theta)*(cos(phi)*q-sin(phi)*r)+xi1/m*cos(phi)*sin(psi)*sin(theta)*(sin(phi)/cos(theta)*q+cos(phi)/cos(theta)*r)-2*xi1/m*cos(phi)*sin(psi)*cos(theta)*(sin(phi)/cos(theta)^2*q*sin(theta)+cos(phi)/cos(theta)^2*r*sin(theta))+xi1/m*(-cos(phi)*sin(psi)*sin(theta)+cos(psi)*sin(phi))*(2*sin(phi)/cos(theta)^3*q*sin(theta)^2+sin(phi)/cos(theta)*q+2*cos(phi)/cos(theta)^3*r*sin(theta)^2+cos(phi)/cos(theta)*r)-1/m*cos(psi)*cos(phi)*sin(theta)*dxi1)*(cos(phi)*q-sin(phi)*r)+(dtran*xi1/m*cos(phi)*sin(psi)*cos(theta)+xi1/m*sin(phi)*sin(psi)*cos(theta)*(p+sin(phi)*tan(theta)*q+cos(phi)*tan(theta)*r)+xi1/m*(cos(psi)*cos(phi)+sin(phi)*sin(psi)*sin(theta))*(sin(phi)*(1+tan(theta)^2)*q+cos(phi)*(1+tan(theta)^2)*r)+xi1/m*sin(psi)*cos(phi)*sin(theta)*(cos(phi)*q-sin(phi)*r)-xi1/m*cos(psi)*cos(phi)*cos(theta)*(sin(phi)/cos(theta)*q+cos(phi)/cos(theta)*r)+xi1/m*(-sin(psi)*sin(phi)-cos(psi)*cos(phi)*sin(theta))*(sin(phi)/cos(theta)^2*q*sin(theta)+cos(phi)/cos(theta)^2*r*sin(theta))-1/m*cos(phi)*sin(psi)*cos(theta)*dxi1)*(sin(phi)/cos(theta)*q+cos(phi)/cos(theta)*r)+(-dtran*xi1/m*(-cos(phi)*sin(psi)*sin(theta)+cos(psi)*sin(phi))+xi1/m*(cos(psi)*cos(phi)+sin(phi)*sin(psi)*sin(theta))*(p+sin(phi)*tan(theta)*q+cos(phi)*tan(theta)*r)-xi1/m*sin(psi)*cos(phi)*cos(theta)*(cos(phi)*q-sin(phi)*r)+xi1/m*(-sin(psi)*sin(phi)-cos(psi)*cos(phi)*sin(theta))*(sin(phi)/cos(theta)*q+cos(phi)/cos(theta)*r)+1/m*(-cos(phi)*sin(psi)*sin(theta)+cos(psi)*sin(phi))*dxi1)*(sin(phi)/cos(theta)^2*q*sin(theta)+cos(phi)/cos(theta)^2*r*sin(theta))-xi1/m*cos(psi)*sin(phi)*cos(theta)*(-drot*p-1/Ixx*(q*Izz*r-r*Iyy*q)+xi2/Ixx)+(-xi1/m*cos(psi)*sin(phi)^2*cos(theta)*tan(theta)+xi1/m*(sin(psi)*cos(phi)-cos(psi)*sin(phi)*sin(theta))*sin(phi)*(1+tan(theta)^2)-xi1/m*cos(phi)^2*cos(psi)*sin(theta)-xi1/m*cos(phi)*sin(psi)*sin(phi)+xi1/m*(-cos(phi)*sin(psi)*sin(theta)+cos(psi)*sin(phi))*sin(phi)/cos(theta)^2*sin(theta))*(-drot*q-1/Iyy*(r*Ixx*p-p*Izz*r)+xi3/Iyy)+(-xi1/m*cos(psi)*sin(phi)*cos(theta)*cos(phi)*tan(theta)+xi1/m*(sin(psi)*cos(phi)-cos(psi)*sin(phi)*sin(theta))*cos(phi)*(1+tan(theta)^2)+xi1/m*cos(phi)*cos(psi)*sin(theta)*sin(phi)-xi1/m*cos(phi)^2*sin(psi)+xi1/m*(-cos(phi)*sin(psi)*sin(theta)+cos(psi)*sin(phi))*cos(phi)/cos(theta)^2*sin(theta))*(-drot*r-1/Izz*(p*Iyy*q-q*Ixx*p)+xi4/Izz)+(-dtran/m*cos(psi)*cos(phi)*cos(theta)-1/m*cos(psi)*sin(phi)*cos(theta)*(p+sin(phi)*tan(theta)*q+cos(phi)*tan(theta)*r)+1/m*(sin(psi)*cos(phi)-cos(psi)*sin(phi)*sin(theta))*(sin(phi)*(1+tan(theta)^2)*q+cos(phi)*(1+tan(theta)^2)*r)-1/m*cos(psi)*cos(phi)*sin(theta)*(cos(phi)*q-sin(phi)*r)-1/m*cos(phi)*sin(psi)*cos(theta)*(sin(phi)/cos(theta)*q+cos(phi)/cos(theta)*r)+1/m*(-cos(phi)*sin(psi)*sin(theta)+cos(psi)*sin(phi))*(sin(phi)/cos(theta)^2*q*sin(theta)+cos(phi)/cos(theta)^2*r*sin(theta)))*dxi1+1/m*cos(psi)*cos(phi)*cos(theta)*ddxi1)*(cos(phi)*q-sin(phi)*r)+(dtran^2*xi1/m*(-cos(phi)*sin(psi)*sin(theta)+cos(psi)*sin(phi))+(-dtran*xi1/m*(cos(psi)*cos(phi)+sin(phi)*sin(psi)*sin(theta))+xi1/m*(cos(phi)*sin(psi)*sin(theta)-cos(psi)*sin(phi))*(p+sin(phi)*tan(theta)*q+cos(phi)*tan(theta)*r)+xi1/m*(cos(psi)*cos(phi)+sin(phi)*sin(psi)*sin(theta))*(cos(phi)*tan(theta)*q-sin(phi)*tan(theta)*r)+xi1/m*sin(psi)*sin(phi)*cos(theta)*(cos(phi)*q-sin(phi)*r)-xi1/m*sin(psi)*cos(phi)*cos(theta)*(-sin(phi)*q-cos(phi)*r)+xi1/m*(cos(psi)*sin(phi)*sin(theta)-sin(psi)*cos(phi))*(sin(phi)/cos(theta)*q+cos(phi)/cos(theta)*r)+xi1/m*(-sin(psi)*sin(phi)-cos(psi)*cos(phi)*sin(theta))*(cos(phi)/cos(theta)*q-sin(phi)/cos(theta)*r)+1/m*(cos(psi)*cos(phi)+sin(phi)*sin(psi)*sin(theta))*dxi1)*(p+sin(phi)*tan(theta)*q+cos(phi)*tan(theta)*r)+(dtran*xi1/m*cos(phi)*sin(psi)*cos(theta)+xi1/m*sin(phi)*sin(psi)*cos(theta)*(p+sin(phi)*tan(theta)*q+cos(phi)*tan(theta)*r)+xi1/m*(cos(psi)*cos(phi)+sin(phi)*sin(psi)*sin(theta))*(sin(phi)*(1+tan(theta)^2)*q+cos(phi)*(1+tan(theta)^2)*r)+xi1/m*sin(psi)*cos(phi)*sin(theta)*(cos(phi)*q-sin(phi)*r)-xi1/m*cos(psi)*cos(phi)*cos(theta)*(sin(phi)/cos(theta)*q+cos(phi)/cos(theta)*r)+xi1/m*(-sin(psi)*sin(phi)-cos(psi)*cos(phi)*sin(theta))*(sin(phi)/cos(theta)^2*q*sin(theta)+cos(phi)/cos(theta)^2*r*sin(theta))-1/m*cos(phi)*sin(psi)*cos(theta)*dxi1)*(cos(phi)*q-sin(phi)*r)+(-dtran*xi1/m*(-sin(psi)*sin(phi)-cos(psi)*cos(phi)*sin(theta))+xi1/m*(cos(psi)*sin(phi)*sin(theta)-sin(psi)*cos(phi))*(p+sin(phi)*tan(theta)*q+cos(phi)*tan(theta)*r)-xi1/m*cos(psi)*cos(phi)*cos(theta)*(cos(phi)*q-sin(phi)*r)+xi1/m*(cos(phi)*sin(psi)*sin(theta)-cos(psi)*sin(phi))*(sin(phi)/cos(theta)*q+cos(phi)/cos(theta)*r)+1/m*(-sin(psi)*sin(phi)-cos(psi)*cos(phi)*sin(theta))*dxi1)*(sin(phi)/cos(theta)*q+cos(phi)/cos(theta)*r)+xi1/m*(cos(psi)*cos(phi)+sin(phi)*sin(psi)*sin(theta))*(-drot*p-1/Ixx*(q*Izz*r-r*Iyy*q)+xi2/Ixx)+(xi1/m*(cos(psi)*cos(phi)+sin(phi)*sin(psi)*sin(theta))*sin(phi)*tan(theta)-xi1/m*cos(phi)^2*sin(psi)*cos(theta)+xi1/m*(-sin(psi)*sin(phi)-cos(psi)*cos(phi)*sin(theta))*sin(phi)/cos(theta))*(-drot*q-1/Iyy*(r*Ixx*p-p*Izz*r)+xi3/Iyy)+(xi1/m*(cos(psi)*cos(phi)+sin(phi)*sin(psi)*sin(theta))*cos(phi)*tan(theta)+xi1/m*cos(phi)*sin(psi)*cos(theta)*sin(phi)+xi1/m*(-sin(psi)*sin(phi)-cos(psi)*cos(phi)*sin(theta))*cos(phi)/cos(theta))*(-drot*r-1/Izz*(p*Iyy*q-q*Ixx*p)+xi4/Izz)+(-dtran/m*(-cos(phi)*sin(psi)*sin(theta)+cos(psi)*sin(phi))+1/m*(cos(psi)*cos(phi)+sin(phi)*sin(psi)*sin(theta))*(p+sin(phi)*tan(theta)*q+cos(phi)*tan(theta)*r)-1/m*sin(psi)*cos(phi)*cos(theta)*(cos(phi)*q-sin(phi)*r)+1/m*(-sin(psi)*sin(phi)-cos(psi)*cos(phi)*sin(theta))*(sin(phi)/cos(theta)*q+cos(phi)/cos(theta)*r))*dxi1+1/m*(-cos(phi)*sin(psi)*sin(theta)+cos(psi)*sin(phi))*ddxi1)*(sin(phi)/cos(theta)*q+cos(phi)/cos(theta)*r)+(2*xi1/m*(-sin(psi)*sin(phi)-cos(psi)*cos(phi)*sin(theta))*(p+sin(phi)*tan(theta)*q+cos(phi)*tan(theta)*r)-dtran*xi1/m*(sin(psi)*cos(phi)-cos(psi)*sin(phi)*sin(theta))+xi1/m*(sin(psi)*cos(phi)-cos(psi)*sin(phi)*sin(theta))*(cos(phi)*tan(theta)*q-sin(phi)*tan(theta)*r)-2*xi1/m*cos(psi)*sin(phi)*cos(theta)*(cos(phi)*q-sin(phi)*r)+xi1/m*cos(psi)*cos(phi)*cos(theta)*(-sin(phi)*q-cos(phi)*r)+2*xi1/m*(cos(psi)*cos(phi)+sin(phi)*sin(psi)*sin(theta))*(sin(phi)/cos(theta)*q+cos(phi)/cos(theta)*r)+xi1/m*(-cos(phi)*sin(psi)*sin(theta)+cos(psi)*sin(phi))*(cos(phi)/cos(theta)*q-sin(phi)/cos(theta)*r)+2/m*(sin(psi)*cos(phi)-cos(psi)*sin(phi)*sin(theta))*dxi1-xi1/m*(sin(psi)*cos(phi)-cos(psi)*sin(phi)*sin(theta))*drot-(xi1/m*(sin(psi)*cos(phi)-cos(psi)*sin(phi)*sin(theta))*sin(phi)*tan(theta)+xi1/m*cos(phi)^2*cos(psi)*cos(theta)+xi1/m*(-cos(phi)*sin(psi)*sin(theta)+cos(psi)*sin(phi))*sin(phi)/cos(theta))/Iyy*(r*Ixx-Izz*r)-(xi1/m*(sin(psi)*cos(phi)-cos(psi)*sin(phi)*sin(theta))*cos(phi)*tan(theta)-xi1/m*cos(phi)*cos(psi)*cos(theta)*sin(phi)+xi1/m*(-cos(phi)*sin(psi)*sin(theta)+cos(psi)*sin(phi))*cos(phi)/cos(theta))/Izz*(Iyy*q-q*Ixx))*(-drot*p-1/Ixx*(q*Izz*r-r*Iyy*q)+xi2/Ixx)+((xi1/m*(-sin(psi)*sin(phi)-cos(psi)*cos(phi)*sin(theta))*sin(phi)*tan(theta)+xi1/m*(sin(psi)*cos(phi)-cos(psi)*sin(phi)*sin(theta))*cos(phi)*tan(theta)-2*xi1/m*cos(phi)*cos(psi)*cos(theta)*sin(phi)+xi1/m*(cos(psi)*cos(phi)+sin(phi)*sin(psi)*sin(theta))*sin(phi)/cos(theta)+xi1/m*(-cos(phi)*sin(psi)*sin(theta)+cos(psi)*sin(phi))*cos(phi)/cos(theta))*(p+sin(phi)*tan(theta)*q+cos(phi)*tan(theta)*r)+(-dtran*xi1/m*(sin(psi)*cos(phi)-cos(psi)*sin(phi)*sin(theta))+xi1/m*(-sin(psi)*sin(phi)-cos(psi)*cos(phi)*sin(theta))*(p+sin(phi)*tan(theta)*q+cos(phi)*tan(theta)*r)+xi1/m*(sin(psi)*cos(phi)-cos(psi)*sin(phi)*sin(theta))*(cos(phi)*tan(theta)*q-sin(phi)*tan(theta)*r)-xi1/m*cos(psi)*sin(phi)*cos(theta)*(cos(phi)*q-sin(phi)*r)+xi1/m*cos(psi)*cos(phi)*cos(theta)*(-sin(phi)*q-cos(phi)*r)+xi1/m*(cos(psi)*cos(phi)+sin(phi)*sin(psi)*sin(theta))*(sin(phi)/cos(theta)*q+cos(phi)/cos(theta)*r)+xi1/m*(-cos(phi)*sin(psi)*sin(theta)+cos(psi)*sin(phi))*(cos(phi)/cos(theta)*q-sin(phi)/cos(theta)*r)+1/m*(sin(psi)*cos(phi)-cos(psi)*sin(phi)*sin(theta))*dxi1)*sin(phi)*tan(theta)+(-xi1/m*cos(psi)*sin(phi)^2*cos(theta)*tan(theta)+xi1/m*(sin(psi)*cos(phi)-cos(psi)*sin(phi)*sin(theta))*sin(phi)*(1+tan(theta)^2)-xi1/m*cos(phi)^2*cos(psi)*sin(theta)-xi1/m*cos(phi)*sin(psi)*sin(phi)+xi1/m*(-cos(phi)*sin(psi)*sin(theta)+cos(psi)*sin(phi))*sin(phi)/cos(theta)^2*sin(theta))*(cos(phi)*q-sin(phi)*r)+(-dtran*xi1/m*cos(psi)*cos(phi)*cos(theta)-xi1/m*cos(psi)*sin(phi)*cos(theta)*(p+sin(phi)*tan(theta)*q+cos(phi)*tan(theta)*r)+xi1/m*(sin(psi)*cos(phi)-cos(psi)*sin(phi)*sin(theta))*(sin(phi)*(1+tan(theta)^2)*q+cos(phi)*(1+tan(theta)^2)*r)-xi1/m*cos(psi)*cos(phi)*sin(theta)*(cos(phi)*q-sin(phi)*r)-xi1/m*cos(phi)*sin(psi)*cos(theta)*(sin(phi)/cos(theta)*q+cos(phi)/cos(theta)*r)+xi1/m*(-cos(phi)*sin(psi)*sin(theta)+cos(psi)*sin(phi))*(sin(phi)/cos(theta)^2*q*sin(theta)+cos(phi)/cos(theta)^2*r*sin(theta))+1/m*cos(psi)*cos(phi)*cos(theta)*dxi1)*cos(phi)+(xi1/m*(cos(psi)*cos(phi)+sin(phi)*sin(psi)*sin(theta))*sin(phi)*tan(theta)-xi1/m*cos(phi)^2*sin(psi)*cos(theta)+xi1/m*(-sin(psi)*sin(phi)-cos(psi)*cos(phi)*sin(theta))*sin(phi)/cos(theta))*(sin(phi)/cos(theta)*q+cos(phi)/cos(theta)*r)+(-dtran*xi1/m*(-cos(phi)*sin(psi)*sin(theta)+cos(psi)*sin(phi))+xi1/m*(cos(psi)*cos(phi)+sin(phi)*sin(psi)*sin(theta))*(p+sin(phi)*tan(theta)*q+cos(phi)*tan(theta)*r)-xi1/m*sin(psi)*cos(phi)*cos(theta)*(cos(phi)*q-sin(phi)*r)+xi1/m*(-sin(psi)*sin(phi)-cos(psi)*cos(phi)*sin(theta))*(sin(phi)/cos(theta)*q+cos(phi)/cos(theta)*r)+1/m*(-cos(phi)*sin(psi)*sin(theta)+cos(psi)*sin(phi))*dxi1)*sin(phi)/cos(theta)-xi1/m*(sin(psi)*cos(phi)-cos(psi)*sin(phi)*sin(theta))/Ixx*(Izz*r-r*Iyy)-(xi1/m*(sin(psi)*cos(phi)-cos(psi)*sin(phi)*sin(theta))*sin(phi)*tan(theta)+xi1/m*cos(phi)^2*cos(psi)*cos(theta)+xi1/m*(-cos(phi)*sin(psi)*sin(theta)+cos(psi)*sin(phi))*sin(phi)/cos(theta))*drot-(xi1/m*(sin(psi)*cos(phi)-cos(psi)*sin(phi)*sin(theta))*cos(phi)*tan(theta)-xi1/m*cos(phi)*cos(psi)*cos(theta)*sin(phi)+xi1/m*(-cos(phi)*sin(psi)*sin(theta)+cos(psi)*sin(phi))*cos(phi)/cos(theta))/Izz*(p*Iyy-Ixx*p)+(1/m*(sin(psi)*cos(phi)-cos(psi)*sin(phi)*sin(theta))*sin(phi)*tan(theta)+1/m*cos(psi)*cos(phi)^2*cos(theta)+1/m*(-cos(phi)*sin(psi)*sin(theta)+cos(psi)*sin(phi))*sin(phi)/cos(theta))*dxi1)*(-drot*q-1/Iyy*(r*Ixx*p-p*Izz*r)+xi3/Iyy)+((xi1/m*(-sin(psi)*sin(phi)-cos(psi)*cos(phi)*sin(theta))*cos(phi)*tan(theta)-xi1/m*(sin(psi)*cos(phi)-cos(psi)*sin(phi)*sin(theta))*sin(phi)*tan(theta)+xi1/m*sin(phi)^2*cos(psi)*cos(theta)-xi1/m*cos(phi)^2*cos(psi)*cos(theta)+xi1/m*(cos(psi)*cos(phi)+sin(phi)*sin(psi)*sin(theta))*cos(phi)/cos(theta)-xi1/m*(-cos(phi)*sin(psi)*sin(theta)+cos(psi)*sin(phi))*sin(phi)/cos(theta))*(p+sin(phi)*tan(theta)*q+cos(phi)*tan(theta)*r)+(-dtran*xi1/m*(sin(psi)*cos(phi)-cos(psi)*sin(phi)*sin(theta))+xi1/m*(-sin(psi)*sin(phi)-cos(psi)*cos(phi)*sin(theta))*(p+sin(phi)*tan(theta)*q+cos(phi)*tan(theta)*r)+xi1/m*(sin(psi)*cos(phi)-cos(psi)*sin(phi)*sin(theta))*(cos(phi)*tan(theta)*q-sin(phi)*tan(theta)*r)-xi1/m*cos(psi)*sin(phi)*cos(theta)*(cos(phi)*q-sin(phi)*r)+xi1/m*cos(psi)*cos(phi)*cos(theta)*(-sin(phi)*q-cos(phi)*r)+xi1/m*(cos(psi)*cos(phi)+sin(phi)*sin(psi)*sin(theta))*(sin(phi)/cos(theta)*q+cos(phi)/cos(theta)*r)+xi1/m*(-cos(phi)*sin(psi)*sin(theta)+cos(psi)*sin(phi))*(cos(phi)/cos(theta)*q-sin(phi)/cos(theta)*r)+1/m*(sin(psi)*cos(phi)-cos(psi)*sin(phi)*sin(theta))*dxi1)*cos(phi)*tan(theta)+(-xi1/m*cos(psi)*sin(phi)*cos(theta)*cos(phi)*tan(theta)+xi1/m*(sin(psi)*cos(phi)-cos(psi)*sin(phi)*sin(theta))*cos(phi)*(1+tan(theta)^2)+xi1/m*cos(phi)*cos(psi)*sin(theta)*sin(phi)-xi1/m*cos(phi)^2*sin(psi)+xi1/m*(-cos(phi)*sin(psi)*sin(theta)+cos(psi)*sin(phi))*cos(phi)/cos(theta)^2*sin(theta))*(cos(phi)*q-sin(phi)*r)-(-dtran*xi1/m*cos(psi)*cos(phi)*cos(theta)-xi1/m*cos(psi)*sin(phi)*cos(theta)*(p+sin(phi)*tan(theta)*q+cos(phi)*tan(theta)*r)+xi1/m*(sin(psi)*cos(phi)-cos(psi)*sin(phi)*sin(theta))*(sin(phi)*(1+tan(theta)^2)*q+cos(phi)*(1+tan(theta)^2)*r)-xi1/m*cos(psi)*cos(phi)*sin(theta)*(cos(phi)*q-sin(phi)*r)-xi1/m*cos(phi)*sin(psi)*cos(theta)*(sin(phi)/cos(theta)*q+cos(phi)/cos(theta)*r)+xi1/m*(-cos(phi)*sin(psi)*sin(theta)+cos(psi)*sin(phi))*(sin(phi)/cos(theta)^2*q*sin(theta)+cos(phi)/cos(theta)^2*r*sin(theta))+1/m*cos(psi)*cos(phi)*cos(theta)*dxi1)*sin(phi)+(xi1/m*(cos(psi)*cos(phi)+sin(phi)*sin(psi)*sin(theta))*cos(phi)*tan(theta)+xi1/m*cos(phi)*sin(psi)*cos(theta)*sin(phi)+xi1/m*(-sin(psi)*sin(phi)-cos(psi)*cos(phi)*sin(theta))*cos(phi)/cos(theta))*(sin(phi)/cos(theta)*q+cos(phi)/cos(theta)*r)+(-dtran*xi1/m*(-cos(phi)*sin(psi)*sin(theta)+cos(psi)*sin(phi))+xi1/m*(cos(psi)*cos(phi)+sin(phi)*sin(psi)*sin(theta))*(p+sin(phi)*tan(theta)*q+cos(phi)*tan(theta)*r)-xi1/m*sin(psi)*cos(phi)*cos(theta)*(cos(phi)*q-sin(phi)*r)+xi1/m*(-sin(psi)*sin(phi)-cos(psi)*cos(phi)*sin(theta))*(sin(phi)/cos(theta)*q+cos(phi)/cos(theta)*r)+1/m*(-cos(phi)*sin(psi)*sin(theta)+cos(psi)*sin(phi))*dxi1)*cos(phi)/cos(theta)-xi1/m*(sin(psi)*cos(phi)-cos(psi)*sin(phi)*sin(theta))/Ixx*(q*Izz-Iyy*q)-(xi1/m*(sin(psi)*cos(phi)-cos(psi)*sin(phi)*sin(theta))*sin(phi)*tan(theta)+xi1/m*cos(phi)^2*cos(psi)*cos(theta)+xi1/m*(-cos(phi)*sin(psi)*sin(theta)+cos(psi)*sin(phi))*sin(phi)/cos(theta))/Iyy*(Ixx*p-p*Izz)-(xi1/m*(sin(psi)*cos(phi)-cos(psi)*sin(phi)*sin(theta))*cos(phi)*tan(theta)-xi1/m*cos(phi)*cos(psi)*cos(theta)*sin(phi)+xi1/m*(-cos(phi)*sin(psi)*sin(theta)+cos(psi)*sin(phi))*cos(phi)/cos(theta))*drot+(1/m*(sin(psi)*cos(phi)-cos(psi)*sin(phi)*sin(theta))*cos(phi)*tan(theta)-1/m*cos(psi)*cos(phi)*cos(theta)*sin(phi)+1/m*(-cos(phi)*sin(psi)*sin(theta)+cos(psi)*sin(phi))*cos(phi)/cos(theta))*dxi1)*(-drot*r-1/Izz*(p*Iyy*q-q*Ixx*p)+xi4/Izz)+(dtran^2/m*(sin(psi)*sin(phi)+cos(psi)*cos(phi)*sin(theta))+(-dtran/m*(sin(psi)*cos(phi)-cos(psi)*sin(phi)*sin(theta))+1/m*(-sin(psi)*sin(phi)-cos(psi)*cos(phi)*sin(theta))*(p+sin(phi)*tan(theta)*q+cos(phi)*tan(theta)*r)+1/m*(sin(psi)*cos(phi)-cos(psi)*sin(phi)*sin(theta))*(cos(phi)*tan(theta)*q-sin(phi)*tan(theta)*r)-1/m*cos(psi)*sin(phi)*cos(theta)*(cos(phi)*q-sin(phi)*r)+1/m*cos(psi)*cos(phi)*cos(theta)*(-sin(phi)*q-cos(phi)*r)+1/m*(cos(psi)*cos(phi)+sin(phi)*sin(psi)*sin(theta))*(sin(phi)/cos(theta)*q+cos(phi)/cos(theta)*r)+1/m*(-cos(phi)*sin(psi)*sin(theta)+cos(psi)*sin(phi))*(cos(phi)/cos(theta)*q-sin(phi)/cos(theta)*r))*(p+sin(phi)*tan(theta)*q+cos(phi)*tan(theta)*r)+(-dtran/m*cos(psi)*cos(phi)*cos(theta)-1/m*cos(psi)*sin(phi)*cos(theta)*(p+sin(phi)*tan(theta)*q+cos(phi)*tan(theta)*r)+1/m*(sin(psi)*cos(phi)-cos(psi)*sin(phi)*sin(theta))*(sin(phi)*(1+tan(theta)^2)*q+cos(phi)*(1+tan(theta)^2)*r)-1/m*cos(psi)*cos(phi)*sin(theta)*(cos(phi)*q-sin(phi)*r)-1/m*cos(phi)*sin(psi)*cos(theta)*(sin(phi)/cos(theta)*q+cos(phi)/cos(theta)*r)+1/m*(-cos(phi)*sin(psi)*sin(theta)+cos(psi)*sin(phi))*(sin(phi)/cos(theta)^2*q*sin(theta)+cos(phi)/cos(theta)^2*r*sin(theta)))*(cos(phi)*q-sin(phi)*r)+(-dtran/m*(-cos(phi)*sin(psi)*sin(theta)+cos(psi)*sin(phi))+1/m*(cos(psi)*cos(phi)+sin(phi)*sin(psi)*sin(theta))*(p+sin(phi)*tan(theta)*q+cos(phi)*tan(theta)*r)-1/m*sin(psi)*cos(phi)*cos(theta)*(cos(phi)*q-sin(phi)*r)+1/m*(-sin(psi)*sin(phi)-cos(psi)*cos(phi)*sin(theta))*(sin(phi)/cos(theta)*q+cos(phi)/cos(theta)*r))*(sin(phi)/cos(theta)*q+cos(phi)/cos(theta)*r)+1/m*(sin(psi)*cos(phi)-cos(psi)*sin(phi)*sin(theta))*(-drot*p-1/Ixx*(q*Izz*r-r*Iyy*q)+xi2/Ixx)+(1/m*(sin(psi)*cos(phi)-cos(psi)*sin(phi)*sin(theta))*sin(phi)*tan(theta)+1/m*cos(psi)*cos(phi)^2*cos(theta)+1/m*(-cos(phi)*sin(psi)*sin(theta)+cos(psi)*sin(phi))*sin(phi)/cos(theta))*(-drot*q-1/Iyy*(r*Ixx*p-p*Izz*r)+xi3/Iyy)+(1/m*(sin(psi)*cos(phi)-cos(psi)*sin(phi)*sin(theta))*cos(phi)*tan(theta)-1/m*cos(psi)*cos(phi)*cos(theta)*sin(phi)+1/m*(-cos(phi)*sin(psi)*sin(theta)+cos(psi)*sin(phi))*cos(phi)/cos(theta))*(-drot*r-1/Izz*(p*Iyy*q-q*Ixx*p)+xi4/Izz))*dxi1+(2/m*(sin(psi)*cos(phi)-cos(psi)*sin(phi)*sin(theta))*(p+sin(phi)*tan(theta)*q+cos(phi)*tan(theta)*r)+2/m*cos(psi)*cos(phi)*cos(theta)*(cos(phi)*q-sin(phi)*r)+2/m*(-cos(phi)*sin(psi)*sin(theta)+cos(psi)*sin(phi))*(sin(phi)/cos(theta)*q+cos(phi)/cos(theta)*r)-dtran/m*(sin(psi)*sin(phi)+cos(psi)*cos(phi)*sin(theta)))*ddxi1;...
% %  -dtran^3*(-dtran*dy+xi1/m*(cos(phi)*sin(psi)*sin(theta)-cos(psi)*sin(phi)))+(dtran^2*xi1/m*(-sin(phi)*sin(psi)*sin(theta)-cos(psi)*cos(phi))+(-dtran*xi1/m*(-cos(phi)*sin(psi)*sin(theta)+cos(psi)*sin(phi))+xi1/m*(sin(phi)*sin(psi)*sin(theta)+cos(psi)*cos(phi))*(p+sin(phi)*tan(theta)*q+cos(phi)*tan(theta)*r)+2*xi1/m*(-cos(phi)*sin(psi)*sin(theta)+cos(psi)*sin(phi))*(cos(phi)*tan(theta)*q-sin(phi)*tan(theta)*r)+xi1/m*(-sin(phi)*sin(psi)*sin(theta)-cos(psi)*cos(phi))*(-sin(phi)*tan(theta)*q-cos(phi)*tan(theta)*r)-xi1/m*cos(phi)*sin(psi)*cos(theta)*(cos(phi)*q-sin(phi)*r)-2*xi1/m*sin(phi)*sin(psi)*cos(theta)*(-sin(phi)*q-cos(phi)*r)+xi1/m*cos(phi)*sin(psi)*cos(theta)*(-cos(phi)*q+sin(phi)*r)+xi1/m*(-sin(psi)*sin(phi)-cos(psi)*cos(phi)*sin(theta))*(sin(phi)/cos(theta)*q+cos(phi)/cos(theta)*r)+2*xi1/m*(sin(psi)*cos(phi)-cos(psi)*sin(phi)*sin(theta))*(cos(phi)/cos(theta)*q-sin(phi)/cos(theta)*r)+xi1/m*(sin(psi)*sin(phi)+cos(psi)*cos(phi)*sin(theta))*(-sin(phi)/cos(theta)*q-cos(phi)/cos(theta)*r)+1/m*(-cos(phi)*sin(psi)*sin(theta)+cos(psi)*sin(phi))*dxi1)*(p+sin(phi)*tan(theta)*q+cos(phi)*tan(theta)*r)+(-dtran*xi1/m*(-sin(phi)*sin(psi)*sin(theta)-cos(psi)*cos(phi))+xi1/m*(-cos(phi)*sin(psi)*sin(theta)+cos(psi)*sin(phi))*(p+sin(phi)*tan(theta)*q+cos(phi)*tan(theta)*r)+xi1/m*(-sin(phi)*sin(psi)*sin(theta)-cos(psi)*cos(phi))*(cos(phi)*tan(theta)*q-sin(phi)*tan(theta)*r)-xi1/m*sin(phi)*sin(psi)*cos(theta)*(cos(phi)*q-sin(phi)*r)+xi1/m*cos(phi)*sin(psi)*cos(theta)*(-sin(phi)*q-cos(phi)*r)+xi1/m*(sin(psi)*cos(phi)-cos(psi)*sin(phi)*sin(theta))*(sin(phi)/cos(theta)*q+cos(phi)/cos(theta)*r)+xi1/m*(sin(psi)*sin(phi)+cos(psi)*cos(phi)*sin(theta))*(cos(phi)/cos(theta)*q-sin(phi)/cos(theta)*r)+1/m*(-sin(phi)*sin(psi)*sin(theta)-cos(psi)*cos(phi))*dxi1)*(cos(phi)*tan(theta)*q-sin(phi)*tan(theta)*r)+(dtran*xi1/m*sin(phi)*sin(psi)*cos(theta)-xi1/m*cos(phi)*sin(psi)*cos(theta)*(p+sin(phi)*tan(theta)*q+cos(phi)*tan(theta)*r)-xi1/m*sin(phi)*sin(psi)*cos(theta)*(cos(phi)*tan(theta)*q-sin(phi)*tan(theta)*r)+xi1/m*(-cos(phi)*sin(psi)*sin(theta)+cos(psi)*sin(phi))*(sin(phi)*(1+tan(theta)^2)*q+cos(phi)*(1+tan(theta)^2)*r)+xi1/m*(-sin(phi)*sin(psi)*sin(theta)-cos(psi)*cos(phi))*(cos(phi)*(1+tan(theta)^2)*q-sin(phi)*(1+tan(theta)^2)*r)+xi1/m*sin(phi)*sin(psi)*sin(theta)*(cos(phi)*q-sin(phi)*r)-xi1/m*cos(phi)*sin(psi)*sin(theta)*(-sin(phi)*q-cos(phi)*r)-xi1/m*cos(psi)*sin(phi)*cos(theta)*(sin(phi)/cos(theta)*q+cos(phi)/cos(theta)*r)+xi1/m*cos(psi)*cos(phi)*cos(theta)*(cos(phi)/cos(theta)*q-sin(phi)/cos(theta)*r)+xi1/m*(sin(psi)*cos(phi)-cos(psi)*sin(phi)*sin(theta))*(sin(phi)/cos(theta)^2*q*sin(theta)+cos(phi)/cos(theta)^2*r*sin(theta))+xi1/m*(sin(psi)*sin(phi)+cos(psi)*cos(phi)*sin(theta))*(cos(phi)/cos(theta)^2*q*sin(theta)-sin(phi)/cos(theta)^2*r*sin(theta))-1/m*sin(phi)*sin(psi)*cos(theta)*dxi1)*(cos(phi)*q-sin(phi)*r)+(-dtran*xi1/m*cos(phi)*sin(psi)*cos(theta)-xi1/m*sin(phi)*sin(psi)*cos(theta)*(p+sin(phi)*tan(theta)*q+cos(phi)*tan(theta)*r)+xi1/m*(-sin(phi)*sin(psi)*sin(theta)-cos(psi)*cos(phi))*(sin(phi)*(1+tan(theta)^2)*q+cos(phi)*(1+tan(theta)^2)*r)-xi1/m*cos(phi)*sin(psi)*sin(theta)*(cos(phi)*q-sin(phi)*r)+xi1/m*cos(psi)*cos(phi)*cos(theta)*(sin(phi)/cos(theta)*q+cos(phi)/cos(theta)*r)+xi1/m*(sin(psi)*sin(phi)+cos(psi)*cos(phi)*sin(theta))*(sin(phi)/cos(theta)^2*q*sin(theta)+cos(phi)/cos(theta)^2*r*sin(theta))+1/m*cos(phi)*sin(psi)*cos(theta)*dxi1)*(-sin(phi)*q-cos(phi)*r)+(-dtran*xi1/m*(sin(psi)*cos(phi)-cos(psi)*sin(phi)*sin(theta))+xi1/m*(-sin(psi)*sin(phi)-cos(psi)*cos(phi)*sin(theta))*(p+sin(phi)*tan(theta)*q+cos(phi)*tan(theta)*r)+xi1/m*(sin(psi)*cos(phi)-cos(psi)*sin(phi)*sin(theta))*(cos(phi)*tan(theta)*q-sin(phi)*tan(theta)*r)-xi1/m*sin(phi)*cos(psi)*cos(theta)*(cos(phi)*q-sin(phi)*r)+xi1/m*cos(phi)*cos(psi)*cos(theta)*(-sin(phi)*q-cos(phi)*r)+xi1/m*(sin(phi)*sin(psi)*sin(theta)+cos(psi)*cos(phi))*(sin(phi)/cos(theta)*q+cos(phi)/cos(theta)*r)+xi1/m*(-cos(phi)*sin(psi)*sin(theta)+cos(psi)*sin(phi))*(cos(phi)/cos(theta)*q-sin(phi)/cos(theta)*r)+1/m*(sin(psi)*cos(phi)-cos(psi)*sin(phi)*sin(theta))*dxi1)*(sin(phi)/cos(theta)*q+cos(phi)/cos(theta)*r)+(-dtran*xi1/m*(sin(psi)*sin(phi)+cos(psi)*cos(phi)*sin(theta))+xi1/m*(sin(psi)*cos(phi)-cos(psi)*sin(phi)*sin(theta))*(p+sin(phi)*tan(theta)*q+cos(phi)*tan(theta)*r)+xi1/m*cos(phi)*cos(psi)*cos(theta)*(cos(phi)*q-sin(phi)*r)+xi1/m*(-cos(phi)*sin(psi)*sin(theta)+cos(psi)*sin(phi))*(sin(phi)/cos(theta)*q+cos(phi)/cos(theta)*r)+1/m*(sin(psi)*sin(phi)+cos(psi)*cos(phi)*sin(theta))*dxi1)*(cos(phi)/cos(theta)*q-sin(phi)/cos(theta)*r)+xi1/m*(-cos(phi)*sin(psi)*sin(theta)+cos(psi)*sin(phi))*(-drot*p-1/Ixx*(q*Izz*r-r*Iyy*q)+xi2/Ixx)+(xi1/m*(-cos(phi)*sin(psi)*sin(theta)+cos(psi)*sin(phi))*sin(phi)*tan(theta)+xi1/m*(-sin(phi)*sin(psi)*sin(theta)-cos(psi)*cos(phi))*cos(phi)*tan(theta)-2*xi1/m*cos(phi)*sin(psi)*cos(theta)*sin(phi)+xi1/m*(sin(psi)*cos(phi)-cos(psi)*sin(phi)*sin(theta))*sin(phi)/cos(theta)+xi1/m*(sin(psi)*sin(phi)+cos(psi)*cos(phi)*sin(theta))*cos(phi)/cos(theta))*(-drot*q-1/Iyy*(r*Ixx*p-p*Izz*r)+xi3/Iyy)+(xi1/m*(-cos(phi)*sin(psi)*sin(theta)+cos(psi)*sin(phi))*cos(phi)*tan(theta)-xi1/m*(-sin(phi)*sin(psi)*sin(theta)-cos(psi)*cos(phi))*sin(phi)*tan(theta)+xi1/m*sin(phi)^2*sin(psi)*cos(theta)-xi1/m*cos(phi)^2*sin(psi)*cos(theta)+xi1/m*(sin(psi)*cos(phi)-cos(psi)*sin(phi)*sin(theta))*cos(phi)/cos(theta)-xi1/m*(sin(psi)*sin(phi)+cos(psi)*cos(phi)*sin(theta))*sin(phi)/cos(theta))*(-drot*r-1/Izz*(p*Iyy*q-q*Ixx*p)+xi4/Izz)+(-dtran/m*(-sin(phi)*sin(psi)*sin(theta)-cos(psi)*cos(phi))+1/m*(-cos(phi)*sin(psi)*sin(theta)+cos(psi)*sin(phi))*(p+sin(phi)*tan(theta)*q+cos(phi)*tan(theta)*r)+1/m*(-sin(phi)*sin(psi)*sin(theta)-cos(psi)*cos(phi))*(cos(phi)*tan(theta)*q-sin(phi)*tan(theta)*r)-1/m*sin(phi)*sin(psi)*cos(theta)*(cos(phi)*q-sin(phi)*r)+1/m*cos(phi)*sin(psi)*cos(theta)*(-sin(phi)*q-cos(phi)*r)+1/m*(sin(psi)*cos(phi)-cos(psi)*sin(phi)*sin(theta))*(sin(phi)/cos(theta)*q+cos(phi)/cos(theta)*r)+1/m*(sin(psi)*sin(phi)+cos(psi)*cos(phi)*sin(theta))*(cos(phi)/cos(theta)*q-sin(phi)/cos(theta)*r))*dxi1+1/m*(-sin(phi)*sin(psi)*sin(theta)-cos(psi)*cos(phi))*ddxi1)*(p+sin(phi)*tan(theta)*q+cos(phi)*tan(theta)*r)+(dtran^2*xi1/m*cos(phi)*sin(psi)*cos(theta)+(dtran*xi1/m*sin(phi)*sin(psi)*cos(theta)-xi1/m*cos(phi)*sin(psi)*cos(theta)*(p+sin(phi)*tan(theta)*q+cos(phi)*tan(theta)*r)-xi1/m*sin(phi)*sin(psi)*cos(theta)*(cos(phi)*tan(theta)*q-sin(phi)*tan(theta)*r)+xi1/m*(-cos(phi)*sin(psi)*sin(theta)+cos(psi)*sin(phi))*(sin(phi)*(1+tan(theta)^2)*q+cos(phi)*(1+tan(theta)^2)*r)+xi1/m*(-sin(phi)*sin(psi)*sin(theta)-cos(psi)*cos(phi))*(cos(phi)*(1+tan(theta)^2)*q-sin(phi)*(1+tan(theta)^2)*r)+xi1/m*sin(phi)*sin(psi)*sin(theta)*(cos(phi)*q-sin(phi)*r)-xi1/m*cos(phi)*sin(psi)*sin(theta)*(-sin(phi)*q-cos(phi)*r)-xi1/m*cos(psi)*sin(phi)*cos(theta)*(sin(phi)/cos(theta)*q+cos(phi)/cos(theta)*r)+xi1/m*cos(psi)*cos(phi)*cos(theta)*(cos(phi)/cos(theta)*q-sin(phi)/cos(theta)*r)+xi1/m*(sin(psi)*cos(phi)-cos(psi)*sin(phi)*sin(theta))*(sin(phi)/cos(theta)^2*q*sin(theta)+cos(phi)/cos(theta)^2*r*sin(theta))+xi1/m*(sin(psi)*sin(phi)+cos(psi)*cos(phi)*sin(theta))*(cos(phi)/cos(theta)^2*q*sin(theta)-sin(phi)/cos(theta)^2*r*sin(theta))-1/m*sin(phi)*sin(psi)*cos(theta)*dxi1)*(p+sin(phi)*tan(theta)*q+cos(phi)*tan(theta)*r)+(-dtran*xi1/m*(-sin(phi)*sin(psi)*sin(theta)-cos(psi)*cos(phi))+xi1/m*(-cos(phi)*sin(psi)*sin(theta)+cos(psi)*sin(phi))*(p+sin(phi)*tan(theta)*q+cos(phi)*tan(theta)*r)+xi1/m*(-sin(phi)*sin(psi)*sin(theta)-cos(psi)*cos(phi))*(cos(phi)*tan(theta)*q-sin(phi)*tan(theta)*r)-xi1/m*sin(phi)*sin(psi)*cos(theta)*(cos(phi)*q-sin(phi)*r)+xi1/m*cos(phi)*sin(psi)*cos(theta)*(-sin(phi)*q-cos(phi)*r)+xi1/m*(sin(psi)*cos(phi)-cos(psi)*sin(phi)*sin(theta))*(sin(phi)/cos(theta)*q+cos(phi)/cos(theta)*r)+xi1/m*(sin(psi)*sin(phi)+cos(psi)*cos(phi)*sin(theta))*(cos(phi)/cos(theta)*q-sin(phi)/cos(theta)*r)+1/m*(-sin(phi)*sin(psi)*sin(theta)-cos(psi)*cos(phi))*dxi1)*(sin(phi)*(1+tan(theta)^2)*q+cos(phi)*(1+tan(theta)^2)*r)+(dtran*xi1/m*cos(phi)*sin(psi)*sin(theta)+xi1/m*sin(phi)*sin(psi)*sin(theta)*(p+sin(phi)*tan(theta)*q+cos(phi)*tan(theta)*r)-2*xi1/m*sin(phi)*sin(psi)*cos(theta)*(sin(phi)*(1+tan(theta)^2)*q+cos(phi)*(1+tan(theta)^2)*r)+xi1/m*(-sin(phi)*sin(psi)*sin(theta)-cos(psi)*cos(phi))*(2*sin(phi)*tan(theta)*(1+tan(theta)^2)*q+2*cos(phi)*tan(theta)*(1+tan(theta)^2)*r)-xi1/m*cos(phi)*sin(psi)*cos(theta)*(cos(phi)*q-sin(phi)*r)-xi1/m*cos(psi)*cos(phi)*sin(theta)*(sin(phi)/cos(theta)*q+cos(phi)/cos(theta)*r)+2*xi1/m*cos(psi)*cos(phi)*cos(theta)*(sin(phi)/cos(theta)^2*q*sin(theta)+cos(phi)/cos(theta)^2*r*sin(theta))+xi1/m*(sin(psi)*sin(phi)+cos(psi)*cos(phi)*sin(theta))*(2*sin(phi)/cos(theta)^3*q*sin(theta)^2+sin(phi)/cos(theta)*q+2*cos(phi)/cos(theta)^3*r*sin(theta)^2+cos(phi)/cos(theta)*r)-1/m*cos(phi)*sin(psi)*sin(theta)*dxi1)*(cos(phi)*q-sin(phi)*r)+(-dtran*xi1/m*cos(psi)*cos(phi)*cos(theta)-xi1/m*cos(psi)*sin(phi)*cos(theta)*(p+sin(phi)*tan(theta)*q+cos(phi)*tan(theta)*r)+xi1/m*(sin(psi)*cos(phi)-cos(psi)*sin(phi)*sin(theta))*(sin(phi)*(1+tan(theta)^2)*q+cos(phi)*(1+tan(theta)^2)*r)-xi1/m*cos(phi)*cos(psi)*sin(theta)*(cos(phi)*q-sin(phi)*r)-xi1/m*cos(phi)*sin(psi)*cos(theta)*(sin(phi)/cos(theta)*q+cos(phi)/cos(theta)*r)+xi1/m*(-cos(phi)*sin(psi)*sin(theta)+cos(psi)*sin(phi))*(sin(phi)/cos(theta)^2*q*sin(theta)+cos(phi)/cos(theta)^2*r*sin(theta))+1/m*cos(psi)*cos(phi)*cos(theta)*dxi1)*(sin(phi)/cos(theta)*q+cos(phi)/cos(theta)*r)+(-dtran*xi1/m*(sin(psi)*sin(phi)+cos(psi)*cos(phi)*sin(theta))+xi1/m*(sin(psi)*cos(phi)-cos(psi)*sin(phi)*sin(theta))*(p+sin(phi)*tan(theta)*q+cos(phi)*tan(theta)*r)+xi1/m*cos(phi)*cos(psi)*cos(theta)*(cos(phi)*q-sin(phi)*r)+xi1/m*(-cos(phi)*sin(psi)*sin(theta)+cos(psi)*sin(phi))*(sin(phi)/cos(theta)*q+cos(phi)/cos(theta)*r)+1/m*(sin(psi)*sin(phi)+cos(psi)*cos(phi)*sin(theta))*dxi1)*(sin(phi)/cos(theta)^2*q*sin(theta)+cos(phi)/cos(theta)^2*r*sin(theta))-xi1/m*sin(phi)*sin(psi)*cos(theta)*(-drot*p-1/Ixx*(q*Izz*r-r*Iyy*q)+xi2/Ixx)+(-xi1/m*sin(phi)^2*sin(psi)*cos(theta)*tan(theta)+xi1/m*(-sin(phi)*sin(psi)*sin(theta)-cos(psi)*cos(phi))*sin(phi)*(1+tan(theta)^2)-xi1/m*cos(phi)^2*sin(psi)*sin(theta)+xi1/m*cos(psi)*cos(phi)*sin(phi)+xi1/m*(sin(psi)*sin(phi)+cos(psi)*cos(phi)*sin(theta))*sin(phi)/cos(theta)^2*sin(theta))*(-drot*q-1/Iyy*(r*Ixx*p-p*Izz*r)+xi3/Iyy)+(-xi1/m*sin(phi)*sin(psi)*cos(theta)*cos(phi)*tan(theta)+xi1/m*(-sin(phi)*sin(psi)*sin(theta)-cos(psi)*cos(phi))*cos(phi)*(1+tan(theta)^2)+xi1/m*cos(phi)*sin(psi)*sin(theta)*sin(phi)+xi1/m*cos(psi)*cos(phi)^2+xi1/m*(sin(psi)*sin(phi)+cos(psi)*cos(phi)*sin(theta))*cos(phi)/cos(theta)^2*sin(theta))*(-drot*r-1/Izz*(p*Iyy*q-q*Ixx*p)+xi4/Izz)+(-dtran/m*cos(phi)*sin(psi)*cos(theta)-1/m*sin(phi)*sin(psi)*cos(theta)*(p+sin(phi)*tan(theta)*q+cos(phi)*tan(theta)*r)+1/m*(-sin(phi)*sin(psi)*sin(theta)-cos(psi)*cos(phi))*(sin(phi)*(1+tan(theta)^2)*q+cos(phi)*(1+tan(theta)^2)*r)-1/m*cos(phi)*sin(psi)*sin(theta)*(cos(phi)*q-sin(phi)*r)+1/m*cos(psi)*cos(phi)*cos(theta)*(sin(phi)/cos(theta)*q+cos(phi)/cos(theta)*r)+1/m*(sin(psi)*sin(phi)+cos(psi)*cos(phi)*sin(theta))*(sin(phi)/cos(theta)^2*q*sin(theta)+cos(phi)/cos(theta)^2*r*sin(theta)))*dxi1+1/m*cos(phi)*sin(psi)*cos(theta)*ddxi1)*(cos(phi)*q-sin(phi)*r)+(dtran^2*xi1/m*(sin(psi)*sin(phi)+cos(psi)*cos(phi)*sin(theta))+(-dtran*xi1/m*(sin(psi)*cos(phi)-cos(psi)*sin(phi)*sin(theta))+xi1/m*(-sin(psi)*sin(phi)-cos(psi)*cos(phi)*sin(theta))*(p+sin(phi)*tan(theta)*q+cos(phi)*tan(theta)*r)+xi1/m*(sin(psi)*cos(phi)-cos(psi)*sin(phi)*sin(theta))*(cos(phi)*tan(theta)*q-sin(phi)*tan(theta)*r)-xi1/m*sin(phi)*cos(psi)*cos(theta)*(cos(phi)*q-sin(phi)*r)+xi1/m*cos(phi)*cos(psi)*cos(theta)*(-sin(phi)*q-cos(phi)*r)+xi1/m*(sin(phi)*sin(psi)*sin(theta)+cos(psi)*cos(phi))*(sin(phi)/cos(theta)*q+cos(phi)/cos(theta)*r)+xi1/m*(-cos(phi)*sin(psi)*sin(theta)+cos(psi)*sin(phi))*(cos(phi)/cos(theta)*q-sin(phi)/cos(theta)*r)+1/m*(sin(psi)*cos(phi)-cos(psi)*sin(phi)*sin(theta))*dxi1)*(p+sin(phi)*tan(theta)*q+cos(phi)*tan(theta)*r)+(-dtran*xi1/m*cos(psi)*cos(phi)*cos(theta)-xi1/m*cos(psi)*sin(phi)*cos(theta)*(p+sin(phi)*tan(theta)*q+cos(phi)*tan(theta)*r)+xi1/m*(sin(psi)*cos(phi)-cos(psi)*sin(phi)*sin(theta))*(sin(phi)*(1+tan(theta)^2)*q+cos(phi)*(1+tan(theta)^2)*r)-xi1/m*cos(phi)*cos(psi)*sin(theta)*(cos(phi)*q-sin(phi)*r)-xi1/m*cos(phi)*sin(psi)*cos(theta)*(sin(phi)/cos(theta)*q+cos(phi)/cos(theta)*r)+xi1/m*(-cos(phi)*sin(psi)*sin(theta)+cos(psi)*sin(phi))*(sin(phi)/cos(theta)^2*q*sin(theta)+cos(phi)/cos(theta)^2*r*sin(theta))+1/m*cos(psi)*cos(phi)*cos(theta)*dxi1)*(cos(phi)*q-sin(phi)*r)+(-dtran*xi1/m*(-cos(phi)*sin(psi)*sin(theta)+cos(psi)*sin(phi))+xi1/m*(sin(phi)*sin(psi)*sin(theta)+cos(psi)*cos(phi))*(p+sin(phi)*tan(theta)*q+cos(phi)*tan(theta)*r)-xi1/m*cos(phi)*sin(psi)*cos(theta)*(cos(phi)*q-sin(phi)*r)+xi1/m*(-sin(psi)*sin(phi)-cos(psi)*cos(phi)*sin(theta))*(sin(phi)/cos(theta)*q+cos(phi)/cos(theta)*r)+1/m*(-cos(phi)*sin(psi)*sin(theta)+cos(psi)*sin(phi))*dxi1)*(sin(phi)/cos(theta)*q+cos(phi)/cos(theta)*r)+xi1/m*(sin(psi)*cos(phi)-cos(psi)*sin(phi)*sin(theta))*(-drot*p-1/Ixx*(q*Izz*r-r*Iyy*q)+xi2/Ixx)+(xi1/m*(sin(psi)*cos(phi)-cos(psi)*sin(phi)*sin(theta))*sin(phi)*tan(theta)+xi1/m*cos(phi)^2*cos(psi)*cos(theta)+xi1/m*(-cos(phi)*sin(psi)*sin(theta)+cos(psi)*sin(phi))*sin(phi)/cos(theta))*(-drot*q-1/Iyy*(r*Ixx*p-p*Izz*r)+xi3/Iyy)+(xi1/m*(sin(psi)*cos(phi)-cos(psi)*sin(phi)*sin(theta))*cos(phi)*tan(theta)-xi1/m*cos(phi)*cos(psi)*cos(theta)*sin(phi)+xi1/m*(-cos(phi)*sin(psi)*sin(theta)+cos(psi)*sin(phi))*cos(phi)/cos(theta))*(-drot*r-1/Izz*(p*Iyy*q-q*Ixx*p)+xi4/Izz)+(-dtran/m*(sin(psi)*sin(phi)+cos(psi)*cos(phi)*sin(theta))+1/m*(sin(psi)*cos(phi)-cos(psi)*sin(phi)*sin(theta))*(p+sin(phi)*tan(theta)*q+cos(phi)*tan(theta)*r)+1/m*cos(phi)*cos(psi)*cos(theta)*(cos(phi)*q-sin(phi)*r)+1/m*(-cos(phi)*sin(psi)*sin(theta)+cos(psi)*sin(phi))*(sin(phi)/cos(theta)*q+cos(phi)/cos(theta)*r))*dxi1+1/m*(sin(psi)*sin(phi)+cos(psi)*cos(phi)*sin(theta))*ddxi1)*(sin(phi)/cos(theta)*q+cos(phi)/cos(theta)*r)+(2*xi1/m*(-cos(phi)*sin(psi)*sin(theta)+cos(psi)*sin(phi))*(p+sin(phi)*tan(theta)*q+cos(phi)*tan(theta)*r)-dtran*xi1/m*(-sin(phi)*sin(psi)*sin(theta)-cos(psi)*cos(phi))+xi1/m*(-sin(phi)*sin(psi)*sin(theta)-cos(psi)*cos(phi))*(cos(phi)*tan(theta)*q-sin(phi)*tan(theta)*r)-2*xi1/m*sin(phi)*sin(psi)*cos(theta)*(cos(phi)*q-sin(phi)*r)+xi1/m*cos(phi)*sin(psi)*cos(theta)*(-sin(phi)*q-cos(phi)*r)+2*xi1/m*(sin(psi)*cos(phi)-cos(psi)*sin(phi)*sin(theta))*(sin(phi)/cos(theta)*q+cos(phi)/cos(theta)*r)+xi1/m*(sin(psi)*sin(phi)+cos(psi)*cos(phi)*sin(theta))*(cos(phi)/cos(theta)*q-sin(phi)/cos(theta)*r)+2/m*(-sin(phi)*sin(psi)*sin(theta)-cos(psi)*cos(phi))*dxi1-xi1/m*(-sin(phi)*sin(psi)*sin(theta)-cos(psi)*cos(phi))*drot-(xi1/m*(-sin(phi)*sin(psi)*sin(theta)-cos(psi)*cos(phi))*sin(phi)*tan(theta)+xi1/m*cos(phi)^2*sin(psi)*cos(theta)+xi1/m*(sin(psi)*sin(phi)+cos(psi)*cos(phi)*sin(theta))*sin(phi)/cos(theta))/Iyy*(r*Ixx-Izz*r)-(xi1/m*(-sin(phi)*sin(psi)*sin(theta)-cos(psi)*cos(phi))*cos(phi)*tan(theta)-xi1/m*cos(phi)*sin(psi)*cos(theta)*sin(phi)+xi1/m*(sin(psi)*sin(phi)+cos(psi)*cos(phi)*sin(theta))*cos(phi)/cos(theta))/Izz*(Iyy*q-q*Ixx))*(-drot*p-1/Ixx*(q*Izz*r-r*Iyy*q)+xi2/Ixx)+((xi1/m*(-cos(phi)*sin(psi)*sin(theta)+cos(psi)*sin(phi))*sin(phi)*tan(theta)+xi1/m*(-sin(phi)*sin(psi)*sin(theta)-cos(psi)*cos(phi))*cos(phi)*tan(theta)-2*xi1/m*cos(phi)*sin(psi)*cos(theta)*sin(phi)+xi1/m*(sin(psi)*cos(phi)-cos(psi)*sin(phi)*sin(theta))*sin(phi)/cos(theta)+xi1/m*(sin(psi)*sin(phi)+cos(psi)*cos(phi)*sin(theta))*cos(phi)/cos(theta))*(p+sin(phi)*tan(theta)*q+cos(phi)*tan(theta)*r)+(-dtran*xi1/m*(-sin(phi)*sin(psi)*sin(theta)-cos(psi)*cos(phi))+xi1/m*(-cos(phi)*sin(psi)*sin(theta)+cos(psi)*sin(phi))*(p+sin(phi)*tan(theta)*q+cos(phi)*tan(theta)*r)+xi1/m*(-sin(phi)*sin(psi)*sin(theta)-cos(psi)*cos(phi))*(cos(phi)*tan(theta)*q-sin(phi)*tan(theta)*r)-xi1/m*sin(phi)*sin(psi)*cos(theta)*(cos(phi)*q-sin(phi)*r)+xi1/m*cos(phi)*sin(psi)*cos(theta)*(-sin(phi)*q-cos(phi)*r)+xi1/m*(sin(psi)*cos(phi)-cos(psi)*sin(phi)*sin(theta))*(sin(phi)/cos(theta)*q+cos(phi)/cos(theta)*r)+xi1/m*(sin(psi)*sin(phi)+cos(psi)*cos(phi)*sin(theta))*(cos(phi)/cos(theta)*q-sin(phi)/cos(theta)*r)+1/m*(-sin(phi)*sin(psi)*sin(theta)-cos(psi)*cos(phi))*dxi1)*sin(phi)*tan(theta)+(-xi1/m*sin(phi)^2*sin(psi)*cos(theta)*tan(theta)+xi1/m*(-sin(phi)*sin(psi)*sin(theta)-cos(psi)*cos(phi))*sin(phi)*(1+tan(theta)^2)-xi1/m*cos(phi)^2*sin(psi)*sin(theta)+xi1/m*cos(psi)*cos(phi)*sin(phi)+xi1/m*(sin(psi)*sin(phi)+cos(psi)*cos(phi)*sin(theta))*sin(phi)/cos(theta)^2*sin(theta))*(cos(phi)*q-sin(phi)*r)+(-dtran*xi1/m*cos(phi)*sin(psi)*cos(theta)-xi1/m*sin(phi)*sin(psi)*cos(theta)*(p+sin(phi)*tan(theta)*q+cos(phi)*tan(theta)*r)+xi1/m*(-sin(phi)*sin(psi)*sin(theta)-cos(psi)*cos(phi))*(sin(phi)*(1+tan(theta)^2)*q+cos(phi)*(1+tan(theta)^2)*r)-xi1/m*cos(phi)*sin(psi)*sin(theta)*(cos(phi)*q-sin(phi)*r)+xi1/m*cos(psi)*cos(phi)*cos(theta)*(sin(phi)/cos(theta)*q+cos(phi)/cos(theta)*r)+xi1/m*(sin(psi)*sin(phi)+cos(psi)*cos(phi)*sin(theta))*(sin(phi)/cos(theta)^2*q*sin(theta)+cos(phi)/cos(theta)^2*r*sin(theta))+1/m*cos(phi)*sin(psi)*cos(theta)*dxi1)*cos(phi)+(xi1/m*(sin(psi)*cos(phi)-cos(psi)*sin(phi)*sin(theta))*sin(phi)*tan(theta)+xi1/m*cos(phi)^2*cos(psi)*cos(theta)+xi1/m*(-cos(phi)*sin(psi)*sin(theta)+cos(psi)*sin(phi))*sin(phi)/cos(theta))*(sin(phi)/cos(theta)*q+cos(phi)/cos(theta)*r)+(-dtran*xi1/m*(sin(psi)*sin(phi)+cos(psi)*cos(phi)*sin(theta))+xi1/m*(sin(psi)*cos(phi)-cos(psi)*sin(phi)*sin(theta))*(p+sin(phi)*tan(theta)*q+cos(phi)*tan(theta)*r)+xi1/m*cos(phi)*cos(psi)*cos(theta)*(cos(phi)*q-sin(phi)*r)+xi1/m*(-cos(phi)*sin(psi)*sin(theta)+cos(psi)*sin(phi))*(sin(phi)/cos(theta)*q+cos(phi)/cos(theta)*r)+1/m*(sin(psi)*sin(phi)+cos(psi)*cos(phi)*sin(theta))*dxi1)*sin(phi)/cos(theta)-xi1/m*(-sin(phi)*sin(psi)*sin(theta)-cos(psi)*cos(phi))/Ixx*(Izz*r-r*Iyy)-(xi1/m*(-sin(phi)*sin(psi)*sin(theta)-cos(psi)*cos(phi))*sin(phi)*tan(theta)+xi1/m*cos(phi)^2*sin(psi)*cos(theta)+xi1/m*(sin(psi)*sin(phi)+cos(psi)*cos(phi)*sin(theta))*sin(phi)/cos(theta))*drot-(xi1/m*(-sin(phi)*sin(psi)*sin(theta)-cos(psi)*cos(phi))*cos(phi)*tan(theta)-xi1/m*cos(phi)*sin(psi)*cos(theta)*sin(phi)+xi1/m*(sin(psi)*sin(phi)+cos(psi)*cos(phi)*sin(theta))*cos(phi)/cos(theta))/Izz*(p*Iyy-Ixx*p)+(1/m*(-sin(phi)*sin(psi)*sin(theta)-cos(psi)*cos(phi))*sin(phi)*tan(theta)+1/m*cos(phi)^2*sin(psi)*cos(theta)+1/m*(sin(psi)*sin(phi)+cos(psi)*cos(phi)*sin(theta))*sin(phi)/cos(theta))*dxi1)*(-drot*q-1/Iyy*(r*Ixx*p-p*Izz*r)+xi3/Iyy)+((xi1/m*(-cos(phi)*sin(psi)*sin(theta)+cos(psi)*sin(phi))*cos(phi)*tan(theta)-xi1/m*(-sin(phi)*sin(psi)*sin(theta)-cos(psi)*cos(phi))*sin(phi)*tan(theta)+xi1/m*sin(phi)^2*sin(psi)*cos(theta)-xi1/m*cos(phi)^2*sin(psi)*cos(theta)+xi1/m*(sin(psi)*cos(phi)-cos(psi)*sin(phi)*sin(theta))*cos(phi)/cos(theta)-xi1/m*(sin(psi)*sin(phi)+cos(psi)*cos(phi)*sin(theta))*sin(phi)/cos(theta))*(p+sin(phi)*tan(theta)*q+cos(phi)*tan(theta)*r)+(-dtran*xi1/m*(-sin(phi)*sin(psi)*sin(theta)-cos(psi)*cos(phi))+xi1/m*(-cos(phi)*sin(psi)*sin(theta)+cos(psi)*sin(phi))*(p+sin(phi)*tan(theta)*q+cos(phi)*tan(theta)*r)+xi1/m*(-sin(phi)*sin(psi)*sin(theta)-cos(psi)*cos(phi))*(cos(phi)*tan(theta)*q-sin(phi)*tan(theta)*r)-xi1/m*sin(phi)*sin(psi)*cos(theta)*(cos(phi)*q-sin(phi)*r)+xi1/m*cos(phi)*sin(psi)*cos(theta)*(-sin(phi)*q-cos(phi)*r)+xi1/m*(sin(psi)*cos(phi)-cos(psi)*sin(phi)*sin(theta))*(sin(phi)/cos(theta)*q+cos(phi)/cos(theta)*r)+xi1/m*(sin(psi)*sin(phi)+cos(psi)*cos(phi)*sin(theta))*(cos(phi)/cos(theta)*q-sin(phi)/cos(theta)*r)+1/m*(-sin(phi)*sin(psi)*sin(theta)-cos(psi)*cos(phi))*dxi1)*cos(phi)*tan(theta)+(-xi1/m*sin(phi)*sin(psi)*cos(theta)*cos(phi)*tan(theta)+xi1/m*(-sin(phi)*sin(psi)*sin(theta)-cos(psi)*cos(phi))*cos(phi)*(1+tan(theta)^2)+xi1/m*cos(phi)*sin(psi)*sin(theta)*sin(phi)+xi1/m*cos(psi)*cos(phi)^2+xi1/m*(sin(psi)*sin(phi)+cos(psi)*cos(phi)*sin(theta))*cos(phi)/cos(theta)^2*sin(theta))*(cos(phi)*q-sin(phi)*r)-(-dtran*xi1/m*cos(phi)*sin(psi)*cos(theta)-xi1/m*sin(phi)*sin(psi)*cos(theta)*(p+sin(phi)*tan(theta)*q+cos(phi)*tan(theta)*r)+xi1/m*(-sin(phi)*sin(psi)*sin(theta)-cos(psi)*cos(phi))*(sin(phi)*(1+tan(theta)^2)*q+cos(phi)*(1+tan(theta)^2)*r)-xi1/m*cos(phi)*sin(psi)*sin(theta)*(cos(phi)*q-sin(phi)*r)+xi1/m*cos(psi)*cos(phi)*cos(theta)*(sin(phi)/cos(theta)*q+cos(phi)/cos(theta)*r)+xi1/m*(sin(psi)*sin(phi)+cos(psi)*cos(phi)*sin(theta))*(sin(phi)/cos(theta)^2*q*sin(theta)+cos(phi)/cos(theta)^2*r*sin(theta))+1/m*cos(phi)*sin(psi)*cos(theta)*dxi1)*sin(phi)+(xi1/m*(sin(psi)*cos(phi)-cos(psi)*sin(phi)*sin(theta))*cos(phi)*tan(theta)-xi1/m*cos(phi)*cos(psi)*cos(theta)*sin(phi)+xi1/m*(-cos(phi)*sin(psi)*sin(theta)+cos(psi)*sin(phi))*cos(phi)/cos(theta))*(sin(phi)/cos(theta)*q+cos(phi)/cos(theta)*r)+(-dtran*xi1/m*(sin(psi)*sin(phi)+cos(psi)*cos(phi)*sin(theta))+xi1/m*(sin(psi)*cos(phi)-cos(psi)*sin(phi)*sin(theta))*(p+sin(phi)*tan(theta)*q+cos(phi)*tan(theta)*r)+xi1/m*cos(phi)*cos(psi)*cos(theta)*(cos(phi)*q-sin(phi)*r)+xi1/m*(-cos(phi)*sin(psi)*sin(theta)+cos(psi)*sin(phi))*(sin(phi)/cos(theta)*q+cos(phi)/cos(theta)*r)+1/m*(sin(psi)*sin(phi)+cos(psi)*cos(phi)*sin(theta))*dxi1)*cos(phi)/cos(theta)-xi1/m*(-sin(phi)*sin(psi)*sin(theta)-cos(psi)*cos(phi))/Ixx*(q*Izz-Iyy*q)-(xi1/m*(-sin(phi)*sin(psi)*sin(theta)-cos(psi)*cos(phi))*sin(phi)*tan(theta)+xi1/m*cos(phi)^2*sin(psi)*cos(theta)+xi1/m*(sin(psi)*sin(phi)+cos(psi)*cos(phi)*sin(theta))*sin(phi)/cos(theta))/Iyy*(Ixx*p-p*Izz)-(xi1/m*(-sin(phi)*sin(psi)*sin(theta)-cos(psi)*cos(phi))*cos(phi)*tan(theta)-xi1/m*cos(phi)*sin(psi)*cos(theta)*sin(phi)+xi1/m*(sin(psi)*sin(phi)+cos(psi)*cos(phi)*sin(theta))*cos(phi)/cos(theta))*drot+(1/m*(-sin(phi)*sin(psi)*sin(theta)-cos(psi)*cos(phi))*cos(phi)*tan(theta)-1/m*cos(phi)*sin(psi)*cos(theta)*sin(phi)+1/m*(sin(psi)*sin(phi)+cos(psi)*cos(phi)*sin(theta))*cos(phi)/cos(theta))*dxi1)*(-drot*r-1/Izz*(p*Iyy*q-q*Ixx*p)+xi4/Izz)+(dtran^2/m*(cos(phi)*sin(psi)*sin(theta)-cos(psi)*sin(phi))+(-dtran/m*(-sin(phi)*sin(psi)*sin(theta)-cos(psi)*cos(phi))+1/m*(-cos(phi)*sin(psi)*sin(theta)+cos(psi)*sin(phi))*(p+sin(phi)*tan(theta)*q+cos(phi)*tan(theta)*r)+1/m*(-sin(phi)*sin(psi)*sin(theta)-cos(psi)*cos(phi))*(cos(phi)*tan(theta)*q-sin(phi)*tan(theta)*r)-1/m*sin(phi)*sin(psi)*cos(theta)*(cos(phi)*q-sin(phi)*r)+1/m*cos(phi)*sin(psi)*cos(theta)*(-sin(phi)*q-cos(phi)*r)+1/m*(sin(psi)*cos(phi)-cos(psi)*sin(phi)*sin(theta))*(sin(phi)/cos(theta)*q+cos(phi)/cos(theta)*r)+1/m*(sin(psi)*sin(phi)+cos(psi)*cos(phi)*sin(theta))*(cos(phi)/cos(theta)*q-sin(phi)/cos(theta)*r))*(p+sin(phi)*tan(theta)*q+cos(phi)*tan(theta)*r)+(-dtran/m*cos(phi)*sin(psi)*cos(theta)-1/m*sin(phi)*sin(psi)*cos(theta)*(p+sin(phi)*tan(theta)*q+cos(phi)*tan(theta)*r)+1/m*(-sin(phi)*sin(psi)*sin(theta)-cos(psi)*cos(phi))*(sin(phi)*(1+tan(theta)^2)*q+cos(phi)*(1+tan(theta)^2)*r)-1/m*cos(phi)*sin(psi)*sin(theta)*(cos(phi)*q-sin(phi)*r)+1/m*cos(psi)*cos(phi)*cos(theta)*(sin(phi)/cos(theta)*q+cos(phi)/cos(theta)*r)+1/m*(sin(psi)*sin(phi)+cos(psi)*cos(phi)*sin(theta))*(sin(phi)/cos(theta)^2*q*sin(theta)+cos(phi)/cos(theta)^2*r*sin(theta)))*(cos(phi)*q-sin(phi)*r)+(-dtran/m*(sin(psi)*sin(phi)+cos(psi)*cos(phi)*sin(theta))+1/m*(sin(psi)*cos(phi)-cos(psi)*sin(phi)*sin(theta))*(p+sin(phi)*tan(theta)*q+cos(phi)*tan(theta)*r)+1/m*cos(phi)*cos(psi)*cos(theta)*(cos(phi)*q-sin(phi)*r)+1/m*(-cos(phi)*sin(psi)*sin(theta)+cos(psi)*sin(phi))*(sin(phi)/cos(theta)*q+cos(phi)/cos(theta)*r))*(sin(phi)/cos(theta)*q+cos(phi)/cos(theta)*r)+1/m*(-sin(phi)*sin(psi)*sin(theta)-cos(psi)*cos(phi))*(-drot*p-1/Ixx*(q*Izz*r-r*Iyy*q)+xi2/Ixx)+(1/m*(-sin(phi)*sin(psi)*sin(theta)-cos(psi)*cos(phi))*sin(phi)*tan(theta)+1/m*cos(phi)^2*sin(psi)*cos(theta)+1/m*(sin(psi)*sin(phi)+cos(psi)*cos(phi)*sin(theta))*sin(phi)/cos(theta))*(-drot*q-1/Iyy*(r*Ixx*p-p*Izz*r)+xi3/Iyy)+(1/m*(-sin(phi)*sin(psi)*sin(theta)-cos(psi)*cos(phi))*cos(phi)*tan(theta)-1/m*cos(phi)*sin(psi)*cos(theta)*sin(phi)+1/m*(sin(psi)*sin(phi)+cos(psi)*cos(phi)*sin(theta))*cos(phi)/cos(theta))*(-drot*r-1/Izz*(p*Iyy*q-q*Ixx*p)+xi4/Izz))*dxi1+(2/m*(-sin(phi)*sin(psi)*sin(theta)-cos(psi)*cos(phi))*(p+sin(phi)*tan(theta)*q+cos(phi)*tan(theta)*r)+2/m*cos(phi)*sin(psi)*cos(theta)*(cos(phi)*q-sin(phi)*r)+2/m*(sin(psi)*sin(phi)+cos(psi)*cos(phi)*sin(theta))*(sin(phi)/cos(theta)*q+cos(phi)/cos(theta)*r)-dtran/m*(cos(phi)*sin(psi)*sin(theta)-cos(psi)*sin(phi)))*ddxi1;...
% % -dtran^3*(-dtran*dz+xi1/m*cos(theta)*cos(phi))+(-dtran^2*xi1/m*cos(theta)*sin(phi)+(dtran*xi1/m*cos(theta)*cos(phi)+xi1/m*cos(theta)*sin(phi)*(p+sin(phi)*tan(theta)*q+cos(phi)*tan(theta)*r)-2*xi1/m*cos(theta)*cos(phi)*(cos(phi)*tan(theta)*q-sin(phi)*tan(theta)*r)-xi1/m*cos(theta)*sin(phi)*(-sin(phi)*tan(theta)*q-cos(phi)*tan(theta)*r)+xi1/m*sin(theta)*cos(phi)*(cos(phi)*q-sin(phi)*r)+2*xi1/m*sin(theta)*sin(phi)*(-sin(phi)*q-cos(phi)*r)-xi1/m*sin(theta)*cos(phi)*(-cos(phi)*q+sin(phi)*r)-1/m*cos(theta)*cos(phi)*dxi1)*(p+sin(phi)*tan(theta)*q+cos(phi)*tan(theta)*r)+(dtran*xi1/m*cos(theta)*sin(phi)-xi1/m*cos(theta)*cos(phi)*(p+sin(phi)*tan(theta)*q+cos(phi)*tan(theta)*r)-xi1/m*cos(theta)*sin(phi)*(cos(phi)*tan(theta)*q-sin(phi)*tan(theta)*r)+xi1/m*sin(theta)*sin(phi)*(cos(phi)*q-sin(phi)*r)-xi1/m*sin(theta)*cos(phi)*(-sin(phi)*q-cos(phi)*r)-1/m*cos(theta)*sin(phi)*dxi1)*(cos(phi)*tan(theta)*q-sin(phi)*tan(theta)*r)+(-dtran*xi1/m*sin(theta)*sin(phi)+xi1/m*sin(theta)*cos(phi)*(p+sin(phi)*tan(theta)*q+cos(phi)*tan(theta)*r)+xi1/m*sin(theta)*sin(phi)*(cos(phi)*tan(theta)*q-sin(phi)*tan(theta)*r)-xi1/m*cos(theta)*cos(phi)*(sin(phi)*(1+tan(theta)^2)*q+cos(phi)*(1+tan(theta)^2)*r)-xi1/m*cos(theta)*sin(phi)*(cos(phi)*(1+tan(theta)^2)*q-sin(phi)*(1+tan(theta)^2)*r)+xi1/m*cos(theta)*sin(phi)*(cos(phi)*q-sin(phi)*r)-xi1/m*cos(theta)*cos(phi)*(-sin(phi)*q-cos(phi)*r)+1/m*sin(theta)*sin(phi)*dxi1)*(cos(phi)*q-sin(phi)*r)+(dtran*xi1/m*sin(theta)*cos(phi)+xi1/m*sin(theta)*sin(phi)*(p+sin(phi)*tan(theta)*q+cos(phi)*tan(theta)*r)-xi1/m*cos(theta)*sin(phi)*(sin(phi)*(1+tan(theta)^2)*q+cos(phi)*(1+tan(theta)^2)*r)-xi1/m*cos(theta)*cos(phi)*(cos(phi)*q-sin(phi)*r)-1/m*sin(theta)*cos(phi)*dxi1)*(-sin(phi)*q-cos(phi)*r)-xi1/m*cos(theta)*cos(phi)*(-drot*p-1/Ixx*(q*Izz*r-r*Iyy*q)+xi2/Ixx)+(-2*xi1/m*cos(theta)*sin(phi)*cos(phi)*tan(theta)+2*xi1/m*sin(theta)*cos(phi)*sin(phi))*(-drot*q-1/Iyy*(r*Ixx*p-p*Izz*r)+xi3/Iyy)+(-xi1/m*cos(theta)*cos(phi)^2*tan(theta)+xi1/m*cos(theta)*sin(phi)^2*tan(theta)-xi1/m*sin(theta)*sin(phi)^2+xi1/m*sin(theta)*cos(phi)^2)*(-drot*r-1/Izz*(p*Iyy*q-q*Ixx*p)+xi4/Izz)+(dtran/m*cos(theta)*sin(phi)-1/m*cos(theta)*cos(phi)*(p+sin(phi)*tan(theta)*q+cos(phi)*tan(theta)*r)-1/m*cos(theta)*sin(phi)*(cos(phi)*tan(theta)*q-sin(phi)*tan(theta)*r)+1/m*sin(theta)*sin(phi)*(cos(phi)*q-sin(phi)*r)-1/m*sin(theta)*cos(phi)*(-sin(phi)*q-cos(phi)*r))*dxi1-1/m*cos(theta)*sin(phi)*ddxi1)*(p+sin(phi)*tan(theta)*q+cos(phi)*tan(theta)*r)+(-dtran^2*xi1/m*sin(theta)*cos(phi)+(-dtran*xi1/m*sin(theta)*sin(phi)+xi1/m*sin(theta)*cos(phi)*(p+sin(phi)*tan(theta)*q+cos(phi)*tan(theta)*r)+xi1/m*sin(theta)*sin(phi)*(cos(phi)*tan(theta)*q-sin(phi)*tan(theta)*r)-xi1/m*cos(theta)*cos(phi)*(sin(phi)*(1+tan(theta)^2)*q+cos(phi)*(1+tan(theta)^2)*r)-xi1/m*cos(theta)*sin(phi)*(cos(phi)*(1+tan(theta)^2)*q-sin(phi)*(1+tan(theta)^2)*r)+xi1/m*cos(theta)*sin(phi)*(cos(phi)*q-sin(phi)*r)-xi1/m*cos(theta)*cos(phi)*(-sin(phi)*q-cos(phi)*r)+1/m*sin(theta)*sin(phi)*dxi1)*(p+sin(phi)*tan(theta)*q+cos(phi)*tan(theta)*r)+(dtran*xi1/m*cos(theta)*sin(phi)-xi1/m*cos(theta)*cos(phi)*(p+sin(phi)*tan(theta)*q+cos(phi)*tan(theta)*r)-xi1/m*cos(theta)*sin(phi)*(cos(phi)*tan(theta)*q-sin(phi)*tan(theta)*r)+xi1/m*sin(theta)*sin(phi)*(cos(phi)*q-sin(phi)*r)-xi1/m*sin(theta)*cos(phi)*(-sin(phi)*q-cos(phi)*r)-1/m*cos(theta)*sin(phi)*dxi1)*(sin(phi)*(1+tan(theta)^2)*q+cos(phi)*(1+tan(theta)^2)*r)+(dtran*xi1/m*cos(theta)*cos(phi)+xi1/m*cos(theta)*sin(phi)*(p+sin(phi)*tan(theta)*q+cos(phi)*tan(theta)*r)+2*xi1/m*sin(theta)*sin(phi)*(sin(phi)*(1+tan(theta)^2)*q+cos(phi)*(1+tan(theta)^2)*r)-xi1/m*cos(theta)*sin(phi)*(2*sin(phi)*tan(theta)*(1+tan(theta)^2)*q+2*cos(phi)*tan(theta)*(1+tan(theta)^2)*r)+xi1/m*sin(theta)*cos(phi)*(cos(phi)*q-sin(phi)*r)-1/m*cos(theta)*cos(phi)*dxi1)*(cos(phi)*q-sin(phi)*r)+xi1/m*sin(theta)*sin(phi)*(-drot*p-1/Ixx*(q*Izz*r-r*Iyy*q)+xi2/Ixx)+(xi1/m*sin(theta)*sin(phi)^2*tan(theta)-xi1/m*cos(theta)*sin(phi)^2*(1+tan(theta)^2)-xi1/m*cos(theta)*cos(phi)^2)*(-drot*q-1/Iyy*(r*Ixx*p-p*Izz*r)+xi3/Iyy)+(xi1/m*sin(theta)*sin(phi)*cos(phi)*tan(theta)-xi1/m*cos(theta)*sin(phi)*cos(phi)*(1+tan(theta)^2)+xi1/m*cos(theta)*cos(phi)*sin(phi))*(-drot*r-1/Izz*(p*Iyy*q-q*Ixx*p)+xi4/Izz)+(dtran/m*sin(theta)*cos(phi)+1/m*sin(theta)*sin(phi)*(p+sin(phi)*tan(theta)*q+cos(phi)*tan(theta)*r)-1/m*cos(theta)*sin(phi)*(sin(phi)*(1+tan(theta)^2)*q+cos(phi)*(1+tan(theta)^2)*r)-1/m*cos(theta)*cos(phi)*(cos(phi)*q-sin(phi)*r))*dxi1-1/m*sin(theta)*cos(phi)*ddxi1)*(cos(phi)*q-sin(phi)*r)+(-2*xi1/m*cos(theta)*cos(phi)*(p+sin(phi)*tan(theta)*q+cos(phi)*tan(theta)*r)+dtran*xi1/m*cos(theta)*sin(phi)-xi1/m*cos(theta)*sin(phi)*(cos(phi)*tan(theta)*q-sin(phi)*tan(theta)*r)+2*xi1/m*sin(theta)*sin(phi)*(cos(phi)*q-sin(phi)*r)-xi1/m*sin(theta)*cos(phi)*(-sin(phi)*q-cos(phi)*r)-2/m*cos(theta)*sin(phi)*dxi1+xi1/m*cos(theta)*sin(phi)*drot-(-xi1/m*cos(theta)*sin(phi)^2*tan(theta)-xi1/m*sin(theta)*cos(phi)^2)/Iyy*(r*Ixx-Izz*r)-(-xi1/m*cos(theta)*sin(phi)*cos(phi)*tan(theta)+xi1/m*sin(theta)*cos(phi)*sin(phi))/Izz*(Iyy*q-q*Ixx))*(-drot*p-1/Ixx*(q*Izz*r-r*Iyy*q)+xi2/Ixx)+((-2*xi1/m*cos(theta)*sin(phi)*cos(phi)*tan(theta)+2*xi1/m*sin(theta)*cos(phi)*sin(phi))*(p+sin(phi)*tan(theta)*q+cos(phi)*tan(theta)*r)+(dtran*xi1/m*cos(theta)*sin(phi)-xi1/m*cos(theta)*cos(phi)*(p+sin(phi)*tan(theta)*q+cos(phi)*tan(theta)*r)-xi1/m*cos(theta)*sin(phi)*(cos(phi)*tan(theta)*q-sin(phi)*tan(theta)*r)+xi1/m*sin(theta)*sin(phi)*(cos(phi)*q-sin(phi)*r)-xi1/m*sin(theta)*cos(phi)*(-sin(phi)*q-cos(phi)*r)-1/m*cos(theta)*sin(phi)*dxi1)*sin(phi)*tan(theta)+(xi1/m*sin(theta)*sin(phi)^2*tan(theta)-xi1/m*cos(theta)*sin(phi)^2*(1+tan(theta)^2)-xi1/m*cos(theta)*cos(phi)^2)*(cos(phi)*q-sin(phi)*r)+(dtran*xi1/m*sin(theta)*cos(phi)+xi1/m*sin(theta)*sin(phi)*(p+sin(phi)*tan(theta)*q+cos(phi)*tan(theta)*r)-xi1/m*cos(theta)*sin(phi)*(sin(phi)*(1+tan(theta)^2)*q+cos(phi)*(1+tan(theta)^2)*r)-xi1/m*cos(theta)*cos(phi)*(cos(phi)*q-sin(phi)*r)-1/m*sin(theta)*cos(phi)*dxi1)*cos(phi)+xi1/m*cos(theta)*sin(phi)/Ixx*(Izz*r-r*Iyy)-(-xi1/m*cos(theta)*sin(phi)^2*tan(theta)-xi1/m*sin(theta)*cos(phi)^2)*drot-(-xi1/m*cos(theta)*sin(phi)*cos(phi)*tan(theta)+xi1/m*sin(theta)*cos(phi)*sin(phi))/Izz*(p*Iyy-Ixx*p)+(-1/m*cos(theta)*sin(phi)^2*tan(theta)-1/m*sin(theta)*cos(phi)^2)*dxi1)*(-drot*q-1/Iyy*(r*Ixx*p-p*Izz*r)+xi3/Iyy)+((-xi1/m*cos(theta)*cos(phi)^2*tan(theta)+xi1/m*cos(theta)*sin(phi)^2*tan(theta)-xi1/m*sin(theta)*sin(phi)^2+xi1/m*sin(theta)*cos(phi)^2)*(p+sin(phi)*tan(theta)*q+cos(phi)*tan(theta)*r)+(dtran*xi1/m*cos(theta)*sin(phi)-xi1/m*cos(theta)*cos(phi)*(p+sin(phi)*tan(theta)*q+cos(phi)*tan(theta)*r)-xi1/m*cos(theta)*sin(phi)*(cos(phi)*tan(theta)*q-sin(phi)*tan(theta)*r)+xi1/m*sin(theta)*sin(phi)*(cos(phi)*q-sin(phi)*r)-xi1/m*sin(theta)*cos(phi)*(-sin(phi)*q-cos(phi)*r)-1/m*cos(theta)*sin(phi)*dxi1)*cos(phi)*tan(theta)+(xi1/m*sin(theta)*sin(phi)*cos(phi)*tan(theta)-xi1/m*cos(theta)*sin(phi)*cos(phi)*(1+tan(theta)^2)+xi1/m*cos(theta)*cos(phi)*sin(phi))*(cos(phi)*q-sin(phi)*r)-(dtran*xi1/m*sin(theta)*cos(phi)+xi1/m*sin(theta)*sin(phi)*(p+sin(phi)*tan(theta)*q+cos(phi)*tan(theta)*r)-xi1/m*cos(theta)*sin(phi)*(sin(phi)*(1+tan(theta)^2)*q+cos(phi)*(1+tan(theta)^2)*r)-xi1/m*cos(theta)*cos(phi)*(cos(phi)*q-sin(phi)*r)-1/m*sin(theta)*cos(phi)*dxi1)*sin(phi)+xi1/m*cos(theta)*sin(phi)/Ixx*(q*Izz-Iyy*q)-(-xi1/m*cos(theta)*sin(phi)^2*tan(theta)-xi1/m*sin(theta)*cos(phi)^2)/Iyy*(Ixx*p-p*Izz)-(-xi1/m*cos(theta)*sin(phi)*cos(phi)*tan(theta)+xi1/m*sin(theta)*cos(phi)*sin(phi))*drot+(-1/m*cos(theta)*sin(phi)*cos(phi)*tan(theta)+1/m*sin(theta)*cos(phi)*sin(phi))*dxi1)*(-drot*r-1/Izz*(p*Iyy*q-q*Ixx*p)+xi4/Izz)+(dtran^2/m*cos(theta)*cos(phi)+(dtran/m*cos(theta)*sin(phi)-1/m*cos(theta)*cos(phi)*(p+sin(phi)*tan(theta)*q+cos(phi)*tan(theta)*r)-1/m*cos(theta)*sin(phi)*(cos(phi)*tan(theta)*q-sin(phi)*tan(theta)*r)+1/m*sin(theta)*sin(phi)*(cos(phi)*q-sin(phi)*r)-1/m*sin(theta)*cos(phi)*(-sin(phi)*q-cos(phi)*r))*(p+sin(phi)*tan(theta)*q+cos(phi)*tan(theta)*r)+(dtran/m*sin(theta)*cos(phi)+1/m*sin(theta)*sin(phi)*(p+sin(phi)*tan(theta)*q+cos(phi)*tan(theta)*r)-1/m*cos(theta)*sin(phi)*(sin(phi)*(1+tan(theta)^2)*q+cos(phi)*(1+tan(theta)^2)*r)-1/m*cos(theta)*cos(phi)*(cos(phi)*q-sin(phi)*r))*(cos(phi)*q-sin(phi)*r)-1/m*cos(theta)*sin(phi)*(-drot*p-1/Ixx*(q*Izz*r-r*Iyy*q)+xi2/Ixx)+(-1/m*cos(theta)*sin(phi)^2*tan(theta)-1/m*sin(theta)*cos(phi)^2)*(-drot*q-1/Iyy*(r*Ixx*p-p*Izz*r)+xi3/Iyy)+(-1/m*cos(theta)*sin(phi)*cos(phi)*tan(theta)+1/m*sin(theta)*cos(phi)*sin(phi))*(-drot*r-1/Izz*(p*Iyy*q-q*Ixx*p)+xi4/Izz))*dxi1+(-2/m*cos(theta)*sin(phi)*(p+sin(phi)*tan(theta)*q+cos(phi)*tan(theta)*r)-2/m*sin(theta)*cos(phi)*(cos(phi)*q-sin(phi)*r)-dtran/m*cos(theta)*cos(phi))*ddxi1;...
% % ((-sin(phi)/cos(theta)*q-cos(phi)/cos(theta)*r)*(p+sin(phi)*tan(theta)*q+cos(phi)*tan(theta)*r)+(cos(phi)/cos(theta)*q-sin(phi)/cos(theta)*r)*(cos(phi)*tan(theta)*q-sin(phi)*tan(theta)*r)+(cos(phi)/cos(theta)^2*q*sin(theta)-sin(phi)/cos(theta)^2*r*sin(theta))*(cos(phi)*q-sin(phi)*r)+(sin(phi)/cos(theta)^2*q*sin(theta)+cos(phi)/cos(theta)^2*r*sin(theta))*(-sin(phi)*q-cos(phi)*r)+cos(phi)/cos(theta)*(-drot*q-1/Iyy*(r*Ixx*p-p*Izz*r)+xi3/Iyy)-sin(phi)/cos(theta)*(-drot*r-1/Izz*(p*Iyy*q-q*Ixx*p)+xi4/Izz))*(p+sin(phi)*tan(theta)*q+cos(phi)*tan(theta)*r)+((cos(phi)/cos(theta)^2*q*sin(theta)-sin(phi)/cos(theta)^2*r*sin(theta))*(p+sin(phi)*tan(theta)*q+cos(phi)*tan(theta)*r)+(cos(phi)/cos(theta)*q-sin(phi)/cos(theta)*r)*(sin(phi)*(1+tan(theta)^2)*q+cos(phi)*(1+tan(theta)^2)*r)+(2*sin(phi)/cos(theta)^3*q*sin(theta)^2+sin(phi)/cos(theta)*q+2*cos(phi)/cos(theta)^3*r*sin(theta)^2+cos(phi)/cos(theta)*r)*(cos(phi)*q-sin(phi)*r)+sin(phi)/cos(theta)^2*(-drot*q-1/Iyy*(r*Ixx*p-p*Izz*r)+xi3/Iyy)*sin(theta)+cos(phi)/cos(theta)^2*(-drot*r-1/Izz*(p*Iyy*q-q*Ixx*p)+xi4/Izz)*sin(theta))*(cos(phi)*q-sin(phi)*r)+(cos(phi)/cos(theta)*q-sin(phi)/cos(theta)*r-sin(phi)/cos(theta)/Iyy*(r*Ixx-Izz*r)-cos(phi)/cos(theta)/Izz*(Iyy*q-q*Ixx))*(-drot*p-1/Ixx*(q*Izz*r-r*Iyy*q)+xi2/Ixx)+(cos(phi)/cos(theta)*(p+sin(phi)*tan(theta)*q+cos(phi)*tan(theta)*r)+(cos(phi)/cos(theta)*q-sin(phi)/cos(theta)*r)*sin(phi)*tan(theta)+sin(phi)/cos(theta)^2*sin(theta)*(cos(phi)*q-sin(phi)*r)+(sin(phi)/cos(theta)^2*q*sin(theta)+cos(phi)/cos(theta)^2*r*sin(theta))*cos(phi)-sin(phi)/cos(theta)*drot-cos(phi)/cos(theta)/Izz*(p*Iyy-Ixx*p))*(-drot*q-1/Iyy*(r*Ixx*p-p*Izz*r)+xi3/Iyy)+(-sin(phi)/cos(theta)*(p+sin(phi)*tan(theta)*q+cos(phi)*tan(theta)*r)+(cos(phi)/cos(theta)*q-sin(phi)/cos(theta)*r)*cos(phi)*tan(theta)+cos(phi)/cos(theta)^2*sin(theta)*(cos(phi)*q-sin(phi)*r)-(sin(phi)/cos(theta)^2*q*sin(theta)+cos(phi)/cos(theta)^2*r*sin(theta))*sin(phi)-sin(phi)/cos(theta)/Iyy*(Ixx*p-p*Izz)-cos(phi)/cos(theta)*drot)*(-drot*r-1/Izz*(p*Iyy*q-q*Ixx*p)+xi4/Izz) ];
% bx = [...
%   dtran^2*(-dtran*dx+xi1/m*(sin(psi)*sin(phi)+cos(psi)*cos(phi)*sin(theta)))+(-dtran*xi1/m*(sin(psi)*cos(phi)-cos(psi)*sin(phi)*sin(theta))+xi1/m*(-sin(psi)*sin(phi)-cos(psi)*cos(phi)*sin(theta))*(p+sin(phi)*tan(theta)*q+cos(phi)*tan(theta)*r)+xi1/m*(sin(psi)*cos(phi)-cos(psi)*sin(phi)*sin(theta))*(cos(phi)*tan(theta)*q-sin(phi)*tan(theta)*r)-xi1/m*cos(psi)*sin(phi)*cos(theta)*(cos(phi)*q-sin(phi)*r)+xi1/m*cos(psi)*cos(phi)*cos(theta)*(-sin(phi)*q-cos(phi)*r)+xi1/m*(sin(phi)*sin(psi)*sin(theta)+cos(psi)*cos(phi))*(sin(phi)/cos(theta)*q+cos(phi)/cos(theta)*r)+xi1/m*(-cos(phi)*sin(psi)*sin(theta)+cos(psi)*sin(phi))*(cos(phi)/cos(theta)*q-sin(phi)/cos(theta)*r)+1/m*(sin(psi)*cos(phi)-cos(psi)*sin(phi)*sin(theta))*dxi1)*(p+sin(phi)*tan(theta)*q+cos(phi)*tan(theta)*r)+(-dtran*xi1/m*cos(psi)*cos(phi)*cos(theta)-xi1/m*cos(psi)*sin(phi)*cos(theta)*(p+sin(phi)*tan(theta)*q+cos(phi)*tan(theta)*r)+xi1/m*(sin(psi)*cos(phi)-cos(psi)*sin(phi)*sin(theta))*(sin(phi)*(1+tan(theta)^2)*q+cos(phi)*(1+tan(theta)^2)*r)-xi1/m*cos(psi)*cos(phi)*sin(theta)*(cos(phi)*q-sin(phi)*r)-xi1/m*cos(phi)*sin(psi)*cos(theta)*(sin(phi)/cos(theta)*q+cos(phi)/cos(theta)*r)+xi1/m*(-cos(phi)*sin(psi)*sin(theta)+cos(psi)*sin(phi))*(sin(phi)/cos(theta)^2*q*sin(theta)+cos(phi)/cos(theta)^2*r*sin(theta))+1/m*cos(psi)*cos(phi)*cos(theta)*dxi1)*(cos(phi)*q-sin(phi)*r)+(-dtran*xi1/m*(-cos(phi)*sin(psi)*sin(theta)+cos(psi)*sin(phi))+xi1/m*(sin(phi)*sin(psi)*sin(theta)+cos(psi)*cos(phi))*(p+sin(phi)*tan(theta)*q+cos(phi)*tan(theta)*r)-xi1/m*sin(psi)*cos(phi)*cos(theta)*(cos(phi)*q-sin(phi)*r)+xi1/m*(-sin(psi)*sin(phi)-cos(psi)*cos(phi)*sin(theta))*(sin(phi)/cos(theta)*q+cos(phi)/cos(theta)*r)+1/m*(-cos(phi)*sin(psi)*sin(theta)+cos(psi)*sin(phi))*dxi1)*(sin(phi)/cos(theta)*q+cos(phi)/cos(theta)*r)+xi1/m*(sin(psi)*cos(phi)-cos(psi)*sin(phi)*sin(theta))*(-drot*p-1/Ixx*(q*Izz*r-r*Iyy*q))+(xi1/m*(sin(psi)*cos(phi)-cos(psi)*sin(phi)*sin(theta))*sin(phi)*tan(theta)+xi1/m*cos(psi)*cos(phi)^2*cos(theta)+xi1/m*(-cos(phi)*sin(psi)*sin(theta)+cos(psi)*sin(phi))*sin(phi)/cos(theta))*(-drot*q-1/Iyy*(r*Ixx*p-p*Izz*r))+(xi1/m*(sin(psi)*cos(phi)-cos(psi)*sin(phi)*sin(theta))*cos(phi)*tan(theta)-xi1/m*cos(psi)*cos(phi)*cos(theta)*sin(phi)+xi1/m*(-cos(phi)*sin(psi)*sin(theta)+cos(psi)*sin(phi))*cos(phi)/cos(theta))*(-drot*r-1/Izz*(p*Iyy*q-q*Ixx*p))+(-dtran/m*(sin(psi)*sin(phi)+cos(psi)*cos(phi)*sin(theta))+1/m*(sin(psi)*cos(phi)-cos(psi)*sin(phi)*sin(theta))*(p+sin(phi)*tan(theta)*q+cos(phi)*tan(theta)*r)+1/m*cos(psi)*cos(phi)*cos(theta)*(cos(phi)*q-sin(phi)*r)+1/m*(-cos(phi)*sin(psi)*sin(theta)+cos(psi)*sin(phi))*(sin(phi)/cos(theta)*q+cos(phi)/cos(theta)*r))*dxi1;...
% dtran^2*(-dtran*dy+xi1/m*(cos(phi)*sin(psi)*sin(theta)-cos(psi)*sin(phi)))+(-dtran*xi1/m*(-sin(phi)*sin(psi)*sin(theta)-cos(psi)*cos(phi))+xi1/m*(-cos(phi)*sin(psi)*sin(theta)+cos(psi)*sin(phi))*(p+sin(phi)*tan(theta)*q+cos(phi)*tan(theta)*r)+xi1/m*(-sin(phi)*sin(psi)*sin(theta)-cos(psi)*cos(phi))*(cos(phi)*tan(theta)*q-sin(phi)*tan(theta)*r)-xi1/m*sin(psi)*sin(phi)*cos(theta)*(cos(phi)*q-sin(phi)*r)+xi1/m*sin(psi)*cos(phi)*cos(theta)*(-sin(phi)*q-cos(phi)*r)+xi1/m*(sin(psi)*cos(phi)-cos(psi)*sin(phi)*sin(theta))*(sin(phi)/cos(theta)*q+cos(phi)/cos(theta)*r)+xi1/m*(sin(psi)*sin(phi)+cos(psi)*cos(phi)*sin(theta))*(cos(phi)/cos(theta)*q-sin(phi)/cos(theta)*r)+1/m*(-sin(phi)*sin(psi)*sin(theta)-cos(psi)*cos(phi))*dxi1)*(p+sin(phi)*tan(theta)*q+cos(phi)*tan(theta)*r)+(-dtran*xi1/m*cos(phi)*sin(psi)*cos(theta)-xi1/m*sin(phi)*sin(psi)*cos(theta)*(p+sin(phi)*tan(theta)*q+cos(phi)*tan(theta)*r)+xi1/m*(-sin(phi)*sin(psi)*sin(theta)-cos(psi)*cos(phi))*(sin(phi)*(1+tan(theta)^2)*q+cos(phi)*(1+tan(theta)^2)*r)-xi1/m*sin(psi)*cos(phi)*sin(theta)*(cos(phi)*q-sin(phi)*r)+xi1/m*cos(psi)*cos(phi)*cos(theta)*(sin(phi)/cos(theta)*q+cos(phi)/cos(theta)*r)+xi1/m*(sin(psi)*sin(phi)+cos(psi)*cos(phi)*sin(theta))*(sin(phi)/cos(theta)^2*q*sin(theta)+cos(phi)/cos(theta)^2*r*sin(theta))+1/m*cos(phi)*sin(psi)*cos(theta)*dxi1)*(cos(phi)*q-sin(phi)*r)+(-dtran*xi1/m*(sin(psi)*sin(phi)+cos(psi)*cos(phi)*sin(theta))+xi1/m*(sin(psi)*cos(phi)-cos(psi)*sin(phi)*sin(theta))*(p+sin(phi)*tan(theta)*q+cos(phi)*tan(theta)*r)+xi1/m*cos(psi)*cos(phi)*cos(theta)*(cos(phi)*q-sin(phi)*r)+xi1/m*(-cos(phi)*sin(psi)*sin(theta)+cos(psi)*sin(phi))*(sin(phi)/cos(theta)*q+cos(phi)/cos(theta)*r)+1/m*(sin(psi)*sin(phi)+cos(psi)*cos(phi)*sin(theta))*dxi1)*(sin(phi)/cos(theta)*q+cos(phi)/cos(theta)*r)+xi1/m*(-sin(phi)*sin(psi)*sin(theta)-cos(psi)*cos(phi))*(-drot*p-1/Ixx*(q*Izz*r-r*Iyy*q))+(xi1/m*(-sin(phi)*sin(psi)*sin(theta)-cos(psi)*cos(phi))*sin(phi)*tan(theta)+xi1/m*sin(psi)*cos(phi)^2*cos(theta)+xi1/m*(sin(psi)*sin(phi)+cos(psi)*cos(phi)*sin(theta))*sin(phi)/cos(theta))*(-drot*q-1/Iyy*(r*Ixx*p-p*Izz*r))+(xi1/m*(-sin(phi)*sin(psi)*sin(theta)-cos(psi)*cos(phi))*cos(phi)*tan(theta)-xi1/m*sin(psi)*cos(phi)*cos(theta)*sin(phi)+xi1/m*(sin(psi)*sin(phi)+cos(psi)*cos(phi)*sin(theta))*cos(phi)/cos(theta))*(-drot*r-1/Izz*(p*Iyy*q-q*Ixx*p))+(-dtran/m*(cos(phi)*sin(psi)*sin(theta)-cos(psi)*sin(phi))+1/m*(-sin(phi)*sin(psi)*sin(theta)-cos(psi)*cos(phi))*(p+sin(phi)*tan(theta)*q+cos(phi)*tan(theta)*r)+1/m*sin(psi)*cos(phi)*cos(theta)*(cos(phi)*q-sin(phi)*r)+1/m*(sin(psi)*sin(phi)+cos(psi)*cos(phi)*sin(theta))*(sin(phi)/cos(theta)*q+cos(phi)/cos(theta)*r))*dxi1;...
% dtran^2*(-dtran*dz-m*g+xi1/m*cos(theta)*cos(phi))+(dtran*xi1/m*cos(theta)*sin(phi)-xi1/m*cos(theta)*cos(phi)*(p+sin(phi)*tan(theta)*q+cos(phi)*tan(theta)*r)-xi1/m*cos(theta)*sin(phi)*(cos(phi)*tan(theta)*q-sin(phi)*tan(theta)*r)+xi1/m*sin(theta)*sin(phi)*(cos(phi)*q-sin(phi)*r)-xi1/m*sin(theta)*cos(phi)*(-sin(phi)*q-cos(phi)*r)-1/m*cos(theta)*sin(phi)*dxi1)*(p+sin(phi)*tan(theta)*q+cos(phi)*tan(theta)*r)+(dtran*xi1/m*sin(theta)*cos(phi)+xi1/m*sin(theta)*sin(phi)*(p+sin(phi)*tan(theta)*q+cos(phi)*tan(theta)*r)-xi1/m*cos(theta)*sin(phi)*(sin(phi)*(1+tan(theta)^2)*q+cos(phi)*(1+tan(theta)^2)*r)-xi1/m*cos(theta)*cos(phi)*(cos(phi)*q-sin(phi)*r)-1/m*sin(theta)*cos(phi)*dxi1)*(cos(phi)*q-sin(phi)*r)-xi1/m*cos(theta)*sin(phi)*(-drot*p-1/Ixx*(q*Izz*r-r*Iyy*q))+(-xi1/m*cos(theta)*sin(phi)^2*tan(theta)-xi1/m*sin(theta)*cos(phi)^2)*(-drot*q-1/Iyy*(r*Ixx*p-p*Izz*r))+(-xi1/m*cos(theta)*sin(phi)*cos(phi)*tan(theta)+xi1/m*sin(theta)*cos(phi)*sin(phi))*(-drot*r-1/Izz*(p*Iyy*q-q*Ixx*p))+(-dtran/m*cos(theta)*cos(phi)-1/m*cos(theta)*sin(phi)*(p+sin(phi)*tan(theta)*q+cos(phi)*tan(theta)*r)-1/m*sin(theta)*cos(phi)*(cos(phi)*q-sin(phi)*r))*dxi1;...
% (cos(phi)/cos(theta)*q-sin(phi)/cos(theta)*r)*(p+sin(phi)*tan(theta)*q+cos(phi)*tan(theta)*r)+(sin(phi)/cos(theta)^2*q*sin(theta)+cos(phi)/cos(theta)^2*r*sin(theta))*(cos(phi)*q-sin(phi)*r)+sin(phi)/cos(theta)*(-drot*q-1/Iyy*(r*Ixx*p-p*Izz*r))+cos(phi)/cos(theta)*(-drot*r-1/Izz*(p*Iyy*q-q*Ixx*p))];
